simulink model "GuytonModel1972_R2018"  (R2018a)
settings: Solver=ode23tb  StartTime=0.0  StopTime=2e6  MaxStep=90  RelTol=1e-3  EnableMultiTasking=on
(part 1 of 2)
settings Model: Creator=Jirka  LastModifiedBy=User
settings SolverCC: ZeroCrossAlgorithm=Adaptive  SolverResetMethod=Robust
settings DataIOCC: LimitDataPoints=on  SaveFormat=Array
settings OptimizationCC: ExpressionDepthLimit=2147483647  InitFltsAndDblsToZero=on  LifeSpan=inf
settings DebuggingCC: SaveWithParameterizedLinksMsg=none  UnderspecifiedInitializationDetection=Classic  MergeDetectMultiDrivingBlocksExec=none  SignalResolutionControl=TryResolveAllWithWarning  MaxConsecutiveZCsMsg=warning  SolverPrmCheckMsg=warning  MultiTaskDSMMsg=warning  MultiTaskCondExecSysMsg=none  FcnCallInpInsideContextMsg=warning  StateNameClashWarn=warning  SFUnexpectedBacktrackingDiag=warning  SFNoUnconditionalDefaultTransitionDiag=warning  SFExecutionAtInitializationDiag=none
settings HardwareCC: ProdBitPerPointer=32  ProdBitPerSizeT=32  ProdBitPerPtrDiffT=32  ProdLargestAtomicFloat=None  ProdIntDivRoundTo=Undefined  ProdEndianess=Unspecified  ProdWordSize=32  ProdHWDeviceType=32-bit Generic
settings ModelReferenceCC: PropagateSignalLabelsOutOfModel=off
settings CodeAppCC: StateflowObjectComments=on
settings GRTTargetCC: TargetFcnLib=ansi_tfl_tmw.mat  TargetLangStandard=C89/C90 (ANSI)  CombineOutputUpdateFcns=off  GRTInterface=on
settings ConfigComp: CovMetricSettings=dw  CovHtmlReporting=on  CovSaveCumulativeToWorkspaceVar=on  CovSaveSingleToWorkspaceVar=on  CovExternalEMLEnable=off

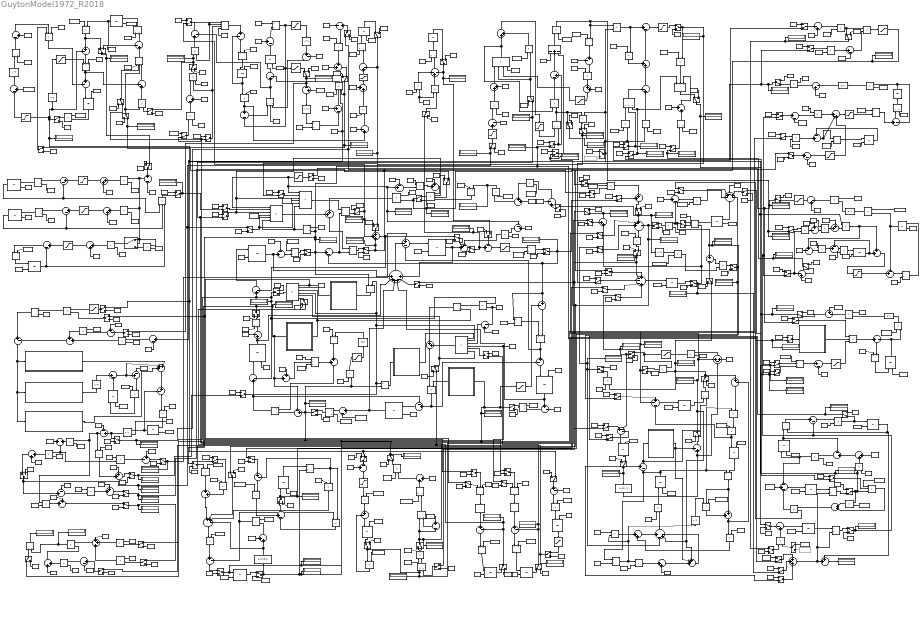
== system GuytonModel1972_R2018 ==
  note: NON-MUSCLE OXYGEN DELIVERY
  note: 269
  note: 268
  note: 261
  note: 260
  note: 270
  note: 262
  note: 263
  note: 264
  note: 271
  note: 272
  note: 265
  note: 266
  note: 267
  note: 259
  note: 258
  note: 257
  note: 256
  note: 255
  note: POV
  note: OSV
  note: POT
  note: RDO
  note: MO2
  note: DOB
  note: QO2
  note: POT
  note: P1O
  note: P4O
  note: 02M
  note: AOM
  note: 271
  note: NON-MUSCLE LOCAL BLOOD FLOW CONTROL
  note: if (POD<0) {POJ=PODx3.3}
  note: 278
  note: 277
  note: 276
  note: 275
  note: 274
  note: 273
  note: 285
  note: 282
  note: 281
  note: 280
  note: 279
  note: 290
  note: 284
  note: 283
  note: 284b
  note: 286
  note: 287
  note: 288
  note: 289
  note: AR1
  note: A1K
  note: POB
  note: POK
  note: POD
  note: POV
  note: ARM
  note: AR1
  note: AR3
  note: PON
  note: POA
  note: A2K
  note: AR2
  note: POJ
  note: POZ
  note: POC
  note: A3K
  note: AR3
  note: POR
  note: VASCULAR
      | STRESS
      | RELAXATION
  note: 65
  note: 64
  note: 63
  note: 62
  note: 61
  note: VV7
  note: VV7
  note: VV1
  note: VV2
  note: VVE
  note: VV6
  note: 195
  note: 196
  note: 197
  note: 198
  note: 199
  note: 200
  note: 201
  note: 202
  note: 203
  note: 205
  note: 206
  note: 207
  note: 208
  note: 209
  note: 210
  note: 211
  note: 212
  note: 213
  note: 214
  note: 215
  note: 216
  note: 217
  note: 218
  note: 219
  note: 220
  note: 221
  note: 222
  note: KIDNEY DYNAMICS AND EXCRETION
  note: THIRST AND DRINKING
  note: 192
  note: 193
  note: 194
  note: 190
  note: 191
  note: STH
  note: TVD
  note: POT
  note: ANTIDIURECTIC HORMONE CONTROL
  note: 181
  note: 180
  note: 179
  note: 178
  note: 177
  note: 175
  note: 176
  note: 182
  note: 183
  note: 184
  note: 185
  note: 158A
  note: 186
  note: 187
  note: 188
  note: 189
  note: AHM
  note: AH4
  note: AH2
  note: AH1
  note: AHC
  note: AH
  note: CNZ
  note: CNA
  note: PRA
  note: AHZ
  note: AH7
  note: AHY
  note: AH8
  note: AU
  note: CIRCULATORY DYNAMICS
  note: VIM
  note: AUM
  note: AUM
  note: VIM
  note: AUM
  note: BFN
  note: 1
  note: 2
  note: 3
  note: 4
  note: 36
  note: 35
  note: 31
  note: 32
  note: 33
  note: PGS
  note: RSM
  note: 38
  note: 34
  note: 37
  note: RVS
  note: 43
  note: 42
  note: 41A
  note: 41
  note: 40
  note: 39
  note: VBD
  note: VVE
  note: 5
  note: 6
  note: 7
  note: 8
  note: 9
  note: DAS
  note: QAO
  note: 30
  note: QLO
  note: LVM
  note: HPL
  note: HMD
  note: QLN
  note: 29
  note: 59
  note: 58
  note: 28
  note: 50
  note: 16
  note: PA2
  note: 60
  note: PLA
  note: 24
  note: 25
  note: 26
  note: 27
  note: VVS
  note: QLO
  note: AUH
  note: HMD
  note: QRO
  note: QRO
  note: AUH
  note: VPE
  note: PPA
  note: PL1
  note: PPA
  note: RPV
  note: RPT
  note: RPT
  note: PP1
  note: 54
  note: 53
  note: 55
  note: 56
  note: 57
  note: 52
  note: 51
  note: 23
  note: 22
  note: 21
  note: 20
  note: 19
  note: 18
  note: 48
  note: 49
  note: 46
  note: 45
  note: 47
  note: 44
  note: 10
  note: 11
  note: 12
  note: 13
  note: 14
  note: 15
  note: LVM
  note: CAPILLARY MEMBRANE DYNAMICS
  note: 66
  note: 67
  note: 68
  note: 69
  note: 70
  note: 71
  note: 74
  note: 73
  note: 82
  note: 81
  note: 80
  note: 79
  note: 78
  note: 77
  note: 75
  note: 76
  note: 72
  note: RVS
  note: BFN
  note: PVG
  note: PVS
  note: VB
  note: VP
  note: VRC
  note: PTC
  note: PPC
  note: PIF
  note: VPD
  note: VUD
  note: DFP
  note: TVD
  note: VP
  note: CPI
  note: CP1
  note: CPP
  note: CPP
  note: PRP
  note: VP
  note: CPR
  note: DLP
  note: PPD
  note: DPL
  note: DPP
  note: DPC
  note: ANGIOTENSIN CONTROL
  note: 154
  note: 157
  note: 158
  note: 159
  note: 160
  note: 161
  note: 162
  note: 163
  note: block 153
  note: block 153
  note: CNA
  note: CNE
  note: ANT
  note: ANC
  note: AN2
  note: AN3
  note: AN5
  note: ANM
  note: REK
  note: GFN
  note: TISSUE FLUIDS, PRESSURES AND GEL
  note: 105
  note: PTC
  note: 108
  note: 107
  note: 106
  note: 109
  note: 104
  note: 110
  note: 103
  note: 102
  note: 112
  note: 113
  note: 98
  note: 97
  note: 96
  note: 99
  note: 92
  note: 91
  note: 90
  note: 89
  note: 93
  note: 94
  note: 95
  note: 100
  note: 101
  note: 86
  note: 85
  note: 84
  note: 83
  note: 87
  note: 88
  note: 111
  note: DPL
  note: VTL
  note: CPI
  note: PIF
  note: PLD
  note: PTT
  note: GP1
  note: GPD
  note: GPR
  note: VG
  note: VIF
  note: PTS
  note: PIF
  note: GPD
  note: DPL
  note: VTC
  note: VTL
  note: VID
  note: VTS
  note: VTD
  note: PTT
  note: DPI
  note: VIF
  note: IFP
  note: GP2
  note: VGD
  note: VG
  note: V2D
  note: PG2
  note: PGC
  note: PTC
  note: PIF
  note: PIF
  note: PTS
  note: PRM
  note: CHY
  note: HYL
  note: VG
  note: PGR
  note: PGP
  note: PGH
  note: ALDOSTERONE CONTROL
  note: 165
  note: 166
  note: 167
  note: 164
  note: 168
  note: 169
  note: 170
  note: 171
  note: 172
  note: 173
  note: 174
  note: AM
  note: AM5
  note: AM3
  note: AM2
  note: AMC
  note: AMT
  note: AM1
  note: AMP
  note: KN1
  note: CKE
  note: CNA
  note: ANM
  note: AMR
  note: ELECTROLYTES AND CELL WATER
  note: 114
  note: 115
  note: 116
  note: 117
  note: 118
  note: 119
  note: 120
  note: 121
  note: 126
  note: 125
  note: 122
  note: 123
  note: 124
  note: 127
  note: 128
  note: 129
  note: 130
  note: 131
  note: 135
  note: 134
  note: 133
  note: 132
  note: CKI
  note: CCD
  note: CNA
  note: VIC
  note: VID
  note: VIC
  note: KI
  note: KCD
  note: KIE
  note: KIR
  note: KE1
  note: AM
  note: CKE
  note: KE
  note: KED
  note: KCD
  note: KID
  note: KOD
  note: REK
  note: NED
  note: NAE
  note: CNA
  note: VTW
  note: VIC
  note: VEC
  note: STH
  note: NID
  note: VP
  note: VPF
  note: VTS
  note: HEART HYPERTROPHY OR DETERIORATION
  note: 340
  note: 341
  note: 342
  note: 343
  note: 344
  note: 349
  note: 348
  note: 347
  note: 346
  note: 345
  note: 350
  note: 351
  note: 352
  note: PA
  note: PPA4
  note: HPL
  note: HPR
  note: PP3
  note: PPA
  note: HSL
  note: HSR
  note: POT
  note: DHM
  note: HMD
  note: RED CELLS AND VISCOSITY
  note: 329
  note: 330
  note: 331
  note: 332
  note: 333
  note: 334
  note: 335
  note: 337
  note: 338
  note: 339
  note: POT
  note: PO2
  note: RC1
  note: RCD
  note: VRC
  note: RKC
  note: RC2
  note: VRC
  note: VB
  note: HM
  note: VIE
  note: VIM
  note: PULMONARY DYNAMICS AND FLUIDS
  note: PLA
  note: 136
  note: 137
  note: 138
  note: 139
  note: 140
  note: 141
  note: 142
  note: 143
  note: 144
  note: 145
  note: 152
  note: 146
  note: 147
  note: 148
  note: 149
  note: 150
  note: 151
  note: PPA
  note: PCP
  note: PPC
  note: POS
  note: PPI
  note: PFI
  note: PLF
  note: DFP
  note: VPF
  note: PPI
  note: PLF
  note: PLF
  note: PPO
  note: POS
  note: CPN
  note: VPF
  note: PPR
  note: PPD
  note: PPN
  note: PPC
  note: CPP
  note: AUTONOMIC CONTROL
  note: 292
  note: 291
  note: 294
  note: 293
  note: 296
  note: 297
  note: 298
  note: 295
  note: 307
  note: 303
  note: 302
  note: 301
  note: 305
  note: 304
  note: 308
  note: 309
  note: 310
  note: 311
  note: 312
  note: 313
  note: 315
  note: 314
  note: 316
  note: 317
  note: 318
  note: 319
  note: 320
  note: POQ
  note: POT
  note: PA
  note: EXE
  note: EX1
  note: P2O
  note: Z12
  note: EXC
  note: AUC
  note: PA1
  note: A1B
  note: AUB
  note: AUN
  note: AU8
  note: AUK
  note: AU2
  note: AU6
  note: DAU
  note: AUJ
  note: AUO
  note: VVR
  note: AUH
  note: AUM
  note: AVE
  note: AUR
  note: AUO
  note: AU9
  note: AU
  note: HEART RATE AND STROKE VOLUME
  note: 328
  note: 327
  note: 323
  note: 322
  note: 321
  note: 324
  note: 325
  note: 326
  note: SVO
  note: QLO
  note: HR
  note: PRA
  note: AUR
  note: HMD
  note: MUSCLE BLOOD FLOW CONTROL AND PO2
  note: 227
  note: 226
  note: 225
  note: 224
  note: 223
  note: 228
  note: 229
  note: 230
  note: 231
  note: 232
  note: 233
  note: 234
  note: 235
  note: 238
  note: 236
  note: 237
  note: 239
  note: 240
  note: 241
  note: 242
  note: 243
  note: 244
  note: 245
  note: 246
  note: 247
  note: 248
  note: 249
  note: 250
  note: 251
  note: 252
  note: 253
  note: 254
  note: OSA
  note: OVA
  note: BFM
  note: RMO
  note: BFM
  note: PK1
  note: PK2
  note: OVS
  note: PVO
  note: PMO
  note: PM5
  note: RMO
  note: QOM
  note: PMO
  note: PM3
  note: PK3
  note: PM4
  note: P2O
  note: P3O
  note: EXC
  note: AOM
  note: O2A
  note: AU
  note: AMM
  note: POE
  note: POM
  note: PDO
  note: PVO
  note: POV
  note: POT
  note: ARM
  note: OVA
  note: P2O
  note: AOM
  note: AMM
  note: AMM
  note: VVE
  note: VV7
  note: VUD
  note: RBF
  note: RFN
  note: NOD
  note: AU
  note: VVR
  note: AUH
  note: AUM
  note: AVE
  note: SVO
  note: HM
  note: BFN
  note: VPF
  note: HM
  note: OVA
  note: PPC
  note: REK
  note: CNE
  note: AUM
  note: AHM
  note: AM
  note: AHM
  note: PA
  note: NOD
  note: DPC
  note: ARM
  note: VIM
  note: AUM
  note: ANM
  note: AVE
  note: RBF
  note: CN3
  note: VVR
  note: VV7
  note: AUH
  note: HMD
  note: HPR
  note: STH
  note: TVD
  note: VTL
  note: AHM
  note: CNE
  note: AM
  note: VID
  note: CKE
  note: CNA
  note: VTW
  note: PC
  note: VB
  note: VP
  note: DPC
  note: CPP
  note: VTC
  note: VTL
  note: DPL
  note: PTC
  note: CPI
  note: VTS
  note: PIF
  note: HPR
  note: HPL
  note: HMD
  note: VIM
  note: HM
  note: VRC
  note: DFP
  note: VPF
  note: PPD
  note: BFN
  note: BFM
  note: RVS
  note: PVS
  note: PRA
  note: QLO
  note: PLA
  note: PPA
  note: PA
  note: HSL
  note: PPC
  note: VTC
  note: PC
  note: GP3
  note: APD
  note: AAR-afferent arteriolar resistance [torr/l/min]
      | AHM-antidiuretic hormone multiplier, ratio of normal effect
      | AM-aldosterone multiplier, ratio of normal effect
      | AMC-aldosterone concentration
      | AMM-muscle vascular constriction caused by local tissue control, ratio to resting state
      | AMP-effect of arterial pressure on rate of aldosterone secretion
      | AMR-effect of sodium to potassium ratio on aldosterone secretion rate
      | AMT-time constant of aldosterone accumulation and destruction
      | ANC-angiotensin concentration
      | ANM-angiotensin multiplier effect on vascular resistance, ratio to normal
      | ANN-effect of sodium concentration on rate of angiotensin formation
      | ANP-effect of renal blood flow on angiotensin formation
      | ANT-time constant of angiotensin accumulation and destruction
      | ANU-nonrenal effect of angiotensin
      | AOM-autonomic effect on tissue oxygen utilization
      | APD-afferent arteriolar pressure drop [torr]
      | ARF-intensity of sympathetic effects on renal function
      | ARM-vasoconstrictor effect of all types of autoregulation
      | AR1-vasoconstrictor effect of rapid autoregulation
      | AR2-vasoconstrictor effects of intermediate autoregulation
      | AR3-vasoconstrictor effect of long-term autoregulation
      | AU-overall activity of autonomic system, ratio to normal
      | AUB-effect of baroreceptors on autoregulation
      | AUC-effect of chemoreceptors on autonomic stimulation
      | AUH-autonomic stimulation of heart, ratio to normal
  note: DLP-rate of formation of plasma protein by liver [g/min]
      | DOB-rate of oxygen delivery to non-muscle cells [ml O2/min]
      | DPA-rate of increase in pulmonary volume [l/min]
      | DPC-rate of loss of plasma proteins through systemic capillaries [g/min]
      | DPI-rate of change of protein in free interstitial fluid [g/min]
      | DPL-rate of systemic lymphatic return of protein [g/min]
      | DPO -rate of loss of plasma protein [g/min]
      | DRA-rate of increase in right atrial volume [l/min]
      | DVS-rate of increase in venous vascular volume [l/min]
      | EVR-postglomerular resistance [torr/l]
      | EXC-exercise activity, ratio to activity at rest
      | EXE-exercise effect on autonomic stimulation
      | GFN-glomerular filtration rate of undamaged kidney [l/min]
      | GFR-glomerular filtration rate [l/min]
      | GLP-glomerular pressure [torr]
      | GPD-rate of increase of protein in gel  [l/min]
      | GPR-total protein in gel  [g]
      | HM-hematocrit [%]
      | HMD-cardiac depressant effect of hypoxia
      | HPL-hypertrophy effect on left ventricle
      | HPR-hypertrophy effect on heart, ratio to normal
      | HR-heart rate [beats/min]
      | HSL-basic left ventricular strength
      | HSR-basic strength of right ventricle
      | HYL-quantity of hyaluronic acid in tissues [g]
      | IFP-interstitial fluid protein [g]
      | KCD-rate of change of potassium concentration [mmol/min]
      | KE-total extracellular fluid potassium [mmol]
      | KED-rate of change of extracellular fluid potassium concentration [mmol/min]
      | KI-total intracellular potassium concentration [mmol/l]
  note: KID-rate of potassium intake [mmol/min]
      | KOD-rate of renal loss of potassium [mmol/min]
      | LVM-effect of aortic pressure on left ventricular output
      | MMO-rate of oxygen utilization by muscle cells [ml/min]
      | M02--rate of oxygen utilization by non-muscle cells [ml/min]
      | NAE-total extracellular sodium [mmol]
      | NED-rate of change of sodium in intracellular fluids [mmol/min]
      | NID-rate of sodium intake [mmol/min]
      | NOD-rate of renal excretion of sodium [mmol/min]
      | OMM-muscle oxygen utilization at rest [ml/min]
      | OSA-aortic oxygen saturation
      | OSV-non-muscle venous oxygen saturation
      | OVA-oxygen volume in aortic blood [ml O2/l blood]
      | OVS-muscle venous oxygen saturation
      | O2M-basic oxygen utilization in non-muscle body tissues [ml/min]
      | PA-aortic pressure  [torr]
      | PAM-effect of arterial pressure in distending arteries, ratio to normal
      | PC-capillary pressure  [torr]
      | PCD-net pressure gradient across capillary membrane  [torr]
      | POP-pulmonary capillary pressure  [torr]
      | PDO-difference between muscle venous oxygen PO2 and normal venous oxygen PO2  [torr]
      | PFI-rate of transfer of fluid across pulmonary capillaries [l/min]
      | PFL-renal filtration pressure  [torr]
      | PGC-colloid osmotic pressure of tissue gel  [torr]
      | PGH-absorbency effect of gel caused by recoil of gel reticulum  [torr]
      | PGL-pressure gradient in lungs  [torr]
      | PGP-colloid osmotic pressure of tissue gel caused by entrapped protein  [torr]
      | PGR-colloid osmotic pressure of interstitial gel caused by Donnan equilibrium  [torr]
      | PIF-interstitial fluid pressure  [torr]
      | PLA-left atrial pressure  [torr]
  note: PLD-pressure gradient to cause lymphatic flow  [torr]
      | PLF-pulmonary lymphatic flow  [torr]
      | PMO-muscle cell PO2  [torr]
      | POD-non-muscle venous PO2 minus normal value  [torr]
      | POK-sensitivity of rapid system of autoregulation
      | PON-sensitivity of intermediate autoregulation
      | POS-pulmonary interstitial fluid colloid osmotic pressure  [torr]
      | POT-non-muscle cell PO2  [torr]
      | POV-non-muscle venous PO2 [torr]
      | POY-sensitivity of red cell production
      | POZ-sensitivity of long-term autoregulation
      | PO2-oxygen deficit factor causing red cell production
      | PPA-pulmonary arterial pressure  [torr]
      | PPC-plasma colloid osmotic pressure  [torr]
      | PPD-rate of change of protein in pulmonary fluids
      | PPI-pulmonary interstitial fluid pressure  [torr]
      | PPN-rate of pulmonary capillary protein loss [g/min]
      | PPO-pulmonary lymph protein flow [g/min]
      | PPR-total protein in pulmonary fluids [g]
      | PRA-right atrial pressure  [torr]
      | PRM-pressure caused by compression of interstitial fluid gel reticulum [torr]
      | PRP-total plasma protein [g]
      | PTC-interstitial fluid colloid osmotic pressure  [torr]
      | PTS-solid tissue pressure  [torr]
      | PTT-total tissue pressure  [torr]
      | PGV-pressure from veins to right atrium  [torr]
      | PVG-venous pressure gradient  [torr]
      | PVO-muscle venous PO2  [torr]
      | PVS-average venous pressure  [torr]
      | QAO-blood flow in the systemic arterial system [l/min]
  note: QLN-basic left ventricular output [l/min]
      | QLO-output of left ventricle [l/min]
      | QOM-total volume of oxygen in muscle cells [ml]
      | QO2-non-muscle total cellular oxygen [ml]
      | QPO-rate of blood flow into pulmonary veins and left atrium [l/min]
      | QRF-feedback effect of left ventricular function on right ventricular function
      | QRN-basic right ventricular output [l/min]
      | QRO-actual right ventricular output [l/min]
      | QVO-rate of blood flow from veins into right atrium [l/min]
      | RAM-basic vascular resistance of muscles [torr/l/min]
      | RAR-basic resistance of non-muscular and non-renal arteries [torr/l/min]
      | RBF-renal blood flow [l/min]
      | RC1-red cell production rate [l/min]
      | RC2-red cell destruction rate [l/min]
      | RCD-rate of change of red cell mass [l/min]
      | REK-percent of normal renal function
      | RFN-renal blood flow if kidney is not damaged [l/min]
      | RKC-rate factor for red cell destruction
      | RM0-rate of oxygen transport to muscle cells [ml/min]
      | RPA-pulmonary arterial resistance [torr/l/min]
      | RPT-pulmonary vascular resistance [torr/l/min]
      | RPV-pulmonary venous resistance [torr/l/min]
      | RR-renal resistance [torr/l/min]
      | RSM-vascular resistance in muscles [torr/l/min]
      | RSN-vascular resistance in non-muscle, non-renal tissues [torr/l/min]
      | RVG-resistance from veins to right atrium [torr/l/min]
      | RVM-depressing effect on right ventricle of pulmonary arterial pressure
      | RVS-venous resistance [torr/l/min]
      | SR-intensity factor for stress relaxation
      | SRK-time constant for stress relaxation
  note: STH-effect of tissue hypoxia on salt and water intake
      | SVO-stroke volume output [l]
      | TRR-tubular reabsorption rate [l/min]
      | TVD-rate of drinking [l/min]
      | VAS-volume in systemic arteries [l]
      | VB-blood volume [l]
      | VEC-extracellular fluid volume [l]
      | VG-volume of interstitial fluid gel [l]
      | VGD-rate of change of tissue gel volumes [l/min]
      | VIB-blood viscosity, ratio to that of water
      | VIC-cell volume [l]
      | VID-rate of fluid transfer between interstitial fluid and cells [l/min]
      | VIE-portion of blood viscosity caused by red blood cells
      | VIF-volume of free interstitial fluid [l]
      | VIM-blood viscosity (ratio to normal blood)
      | VLA-volume in left atrium [l]
      | VP-plasma volume [l]
      | VPA-volume in pulmonary arteries [l]
      | VPD-rate of change of plasma volume [l]
      | VPF-pulmonary free fluid volume [l]
      | VRA-right atrial volume [l]
      | VTC-rate of fluid transfer across systemic capillary membranes [l/min]
      | VTD-rate of volume change in total interstitial fluid [l/min]
      | VTL-rate of systemic lymph flow [l/min]
      | VTW-total body water [l]
      | VUD-rate of urinary output [l/min]
      | VV7-increased vascular volume caused by stress relaxation [l]
      | VVR-diminished vascular volume caused by sympathetic stimulation [l]
      | VVS-venous vascular volume [l]
      | Z8-time constant of autonomic response
  note: AUK-time constant of baroreceptor adaptation
      | AUL-sensitivity of sympathetic control of vascular capacitance
      | AUM-sympathetic vasoconstrictor effect on arteries
      | AUN-effect of CNS ischemic reflex on auto-regulation
      | AUV-sensitivity control of autonomies on heart function
      | AUY-sensitivity of sympathetic control of veins
      | AUZ-overall sensitivity of autonomic control
      | AVE-sympathetic vasoconstrictor effect on veins
      | AlK-time constant of rapid autoregulation
      | A2K-time constant of intermediate autoregulation
      | A3K-time constant of long-term autoregulation
      | A4K-time constant for muscle local vascular response to metabolic activity
      | BFM-muscle blood flow [l/min]
      | BFN-blood flow in non-muscle, non-renal tissues [l/min]
      | CA-capacitance of systemic arteries [l/torr]
      | CCD-concentration gradient across cell membrane [mmol/l]
      | CHY-concentration of hyaluronic acid in tissue fluids [g/l]
      | CKE-extracellular potassium concentration [mmol/l]
      | CKI-intracellular potassium concentration [mmol/l]
      | CNA-extracellular sodium concentration [mmol/l]
      | CNE-sodium concentration abnormality causing third factor effect [mmo/l]
      | CPG-concentration of protein in tissue gel [g/l]
      | CPI-concentration of protein in free interstitial fluid [g/l]
      | CPN-concentration of protein in pulmonary fluids [g/l]
      | CPP-plasma protein concentration [g/l]
      | CV-venous capacitance [l/torr]
      | DAS-rate of volume increase of systemic arteries [l/min]
      | DFP-rate of increase in pulmonary free fluid [l/min]
      | DHM-rate of cardiac deterioration caused by hypoxia
      | DLA-rate of volume increase in pulmonary veins and left atrium [l/min]
  note: LIST OF VARIABLES
  note: 336
  note: HM2
  note: 336b
  note: HMK
  note: HR
  note: PA
  note: OMM
  note: PA0
  note: 299
  note: 300
  note: 306
  note: HR
  note: HRN
  note: HRPRA
  note: HRAU
  note: HRHMD
  note: HKM
  note: VIB
  note: PVG
  note: RDNORM
  note: 17
  note: DPA
  note: RSNA
  note: RSNV
  note: QRRF
  note: FQLN
  note: FQRN
  note: RVV7
  note: CPPK
  note: LPD
  note: PGH
  note: CPG
  note: PHYX
  note: PGX
  note: PC
  note: VIM
  note: AGK
  note: ANW
  note: ANR
  note: ANV
  note: ANP
  note: AN1
  note: 155-156
  note: AU
  note: AUP
  note: AUR
  note: AUR
  note: 315a
  note: 312B
  note: 312A
  " lower limit 0" : Saturate  UpperLimit=inf  LowerLimit=0.0001  LinearizeAsGain=off
  " lower limit 0.35" : Saturate  UpperLimit=inf  LowerLimit=0.35  LinearizeAsGain=off
   VAS{,1..5} (6 alike) : Integrator  InitialConditionSource=external
  " VLA" : Integrator  InitialConditionSource=external
  " VPA" : Integrator  InitialConditionSource=external
  " VRA" : Integrator  InitialConditionSource=external
  " VVS" : Integrator  InitialConditionSource=external
  "1 " : Constant
  AMP = f(PA) : Subsystem
      mask Display:
      | plot([ 0    10    20    30    40    50    60    70    80    90   100   110   120   130   140   150   160   170   180   190   200], [4.0000    3.6505    3.3040    2.9635    2.6320    2.3125    2.0080    1.7215    1.4560    1.2145    1.0000    0.8145    0.6560    0.5215    0.4080    0.3125    0.2320    0.1635    0.1040    0.0505    0.0000])
      | 
      | text(-20,2,'')
      | text(230,2,'')
      | text(100,4.2,'')
      | text(100,-0.4,'')
      | 
      | text(-16,0,'0')
      | text(0,-0.2,'0')
      | text(-16,4,'4')
      | text(190,-0.2,'200')
  ANY : Constant  Value=0.2
  ANZ : Constant  Value=0.4
  ARF : Constant  Value=1.5
  AUB calculation : Subsystem
      mask Display: disp('AUB CALCULATION \n\nwhen PA1<40: AUB=1.85718             \nwhen  40>PA1<170: AUB=0.014286*(170-PA1)\nwhen PA1>=170: AUB=0               \n')
  AUB^3 : Fcn  Expr=u^3
  AUC calculation : Subsystem
      mask Display: disp('AUC CALCULATION \n\nwhen PA1<40: AUC=1.2             \nwhen  40>PA1<80: AUC=0.03*(80-PA1)\nwhen PA1>=80: AUC=0               \n')
  AUJ^AUZ : Math  Operator=pow  SaturateOnIntegerOverflow=on
  AUL : Constant  Value=0.21
  AUN calculation : Subsystem
      mask Display: disp('AUN CALCULATION \n\nwhen PA1<50: AUN=6            \nwhen  20>PA1<50: AUN=0.2*(50-PA1)\nwhen PA1>=50: AUN=0               \n')
  AUQ : Constant
  AUS : Constant
  AUV : Constant  Value=0.3
  AUY : Constant  Value=0.5
  AUZ : Constant
  CFC : Constant  Value=0.007
  CHY^2 : Fcn  Expr=u^2
  CN2 : Constant  Value=0.0212
  CN7 : Constant  Value=0.2
  CNR : Constant  Value=139
  CNX : Constant  Value=2.5
  CNY : Constant  Value=6
  CPF : Constant  Value=0.0003
  CPK : Constant  Value=1.6283e-007
  CV : Constant  Value=0.0825
  Constant{1,14,16,18..20,22..24,27,29,35,45..47,54,58,61,67,76,78,94,137,149..150,153..155,158,160,166,169,171,175..176,183,189..191,195..196,198..201,205,209,213,216,234..235,241,244..249,254..257,260,274,280,282..283,285,295..297,299,304..306,308..309,322,327..328,330..331,334..335} (84 alike) : Constant
  Constant{7..8,10,172,178,211,229,237,258,267,287,290,315,324} (14 alike) : Constant  Value=5
  Constant100 : Constant  Value=0.013332
  Constant101 : Constant  Value=0.25
  Constant102 : Constant  Value=7.8
  Constant103 : Constant  Value=0.004
  Constant{63..64,85,104,116,215,277} (7 alike) : Constant  Value=0.1
  Constant{82..83,86,105,146} (5 alike) : Constant  Value=0.4
  Constant106 : Constant  Value=57
  Constant107 : Constant  Value=-5.9
  Constant108 : Constant  Value=24.2
  Constant109 : Constant  Value=0.25
  Constant11 : Constant  Value=-1
  Constant110 : Constant  Value=9
  Constant111 : Constant  Value=60
  Constant112 : Constant  Value=-0.0391
  Constant113 : Constant  Value=19.8
  Constant114 : Constant  Value=20.039
  Constant115 : Constant  Value=0.00352
  Constant117 : Constant  Value=0.00042
  Constant118 : Constant  Value=0.00014
  Constant119 : Constant  Value=0.0028
  Constant12 : Constant  Value=8.0001
  Constant120 : Constant  Value=0.013
  Constant121 : Constant  Value=140
  Constant122 : Constant  Value=0.01
  Constant123 : Constant  Value=2850
  Constant{62,124,132,193,210,223,238,323} (8 alike) : Constant  Value=100
  Constant125 : Constant  Value=57600
  Constant{95,126,224,230,326} (5 alike) : Constant  Value=15
  Constant127 : Constant  Value=57600
  Constant128 : Constant  Value=6
  Constant129 : Constant  Value=0.0025
  Constant13 : Constant  Value=512
  Constant131 : Constant  Value=0.0000058
  Constant134 : Constant  Value=0.5333
  Constant135 : Constant  Value=1.5
  Constant136 : Constant  Value=0.333
  Constant138 : Constant  Value=0.55
  Constant{139,187,217,301} (4 alike) : Constant  Value=0.0125
  Constant140 : Constant  Value=0.4667
  Constant142 : Constant  Value=11
  Constant143 : Constant  Value=0.0003
  Constant144 : Constant  Value=0.000225
  Constant145 : Constant  Value=0.375
  Constant{147,157,204,214,226..228,239..240} (9 alike) : Constant  Value=8
  Constant15 : Constant  Value=60
  Constant151 : Constant  Value=0.15
  Constant152 : Constant  Value=0.85
  Constant{56,156,218,310} (4 alike) : Constant  Value=3
  Constant159 : Constant  Value=1.24
  Constant161 : Constant  Value=0.0005
  Constant164 : Constant  Value=2
  Constant{25,165,174,184,188,206,243,300} (8 alike) : Constant  Value=40
  Constant167 : Constant  Value=0.5
  Constant168 : Constant  Value=32
  Constant17 : Constant  Value=0.15
  Constant170 : Constant  Value=0.025
  Constant173 : Constant  Value=0.08
  Constant177 : Constant  Value=0.5
  Constant179 : Constant  Value=57.14
  Constant180 : Constant  Value=122
  Constant181 : Constant  Value=2500
  Constant182 : Constant  Value=800
  Constant185 : Constant  Value=2.8
  Constant186 : Constant  Value=200
  Constant{30..31,192,319} (4 alike) : Constant  Value=0.3
  Constant194 : Constant  Value=28
  Constant{197,284,332..333} (4 alike) : Constant  Value=10
  Constant2 : Constant  Value=168
  Constant{202,221,231,236,253,268,271,275,286,302..303,320,325} (13 alike) : Constant  Value=0
  Constant{203,207,212,288} (4 alike) : Constant  Value=142
  Constant208 : Constant  Value=0.125
  Constant21 : Constant  Value=11520
  Constant219 : Constant  Value=12
  Constant{220,270,291,313} (4 alike) : Constant  Value=0.002
  Constant{222,273,292,312} (4 alike) : Constant  Value=0.04
  Constant225 : Constant  Value=200
  Constant232 : Constant  Value=28
  Constant233 : Constant  Value=70
  Constant250 : Constant  Value=1.2
  Constant{68..69,251,314} (4 alike) : Constant  Value=17
  Constant252 : Constant  Value=2.95
  Constant26 : Constant  Value=0.06
  Constant{38,261,269,276} (4 alike) : Constant  Value=0.001
  Constant262 : Constant  Value=2.9
  Constant263 : Constant  Value=2.8
  Constant264 : Constant  Value=3.7
  Constant265 : Constant  Value=2
  Constant266 : Constant  Value=-6.3
  Constant{28,74,272,294} (4 alike) : Constant  Value=20
  Constant278 : Constant  Value=1.2
  Constant279 : Constant  Value=1.2
  Constant281 : Constant  Value=17.75
  Constant289 : Constant  Value=12
  Constant293 : Constant  Value=-6.3
  Constant298 : Constant  Value=2
  Constant3 : Constant  Value=2688
  Constant307 : Constant  Value=2.95
  Constant311 : Constant  Value=70
  Constant316 : Constant  Value=28
  Constant317 : Constant  Value=3.7
  Constant318 : Constant  Value=2.9
  Constant32 : Constant  Value=0.301
  Constant321 : Constant  Value=2.8
  Constant329 : Constant  Value=0.2
  Constant33 : Constant  Value=0.5
  Constant36 : Constant  Value=0.8
  Constant37 : Constant  Value=1000
  Constant39 : Constant  Value=0.025
  Constant4 : Constant  Value=8.0001
  Constant40 : Constant  Value=31.67
  Constant41 : Constant  Value=51.66
  Constant42 : Constant  Value=18
  Constant43 : Constant  Value=0.00781
  Constant44 : Constant  Value=0.125
  Constant48 : Constant  Value=0.01
  Constant49 : Constant  Value=0.009
  Constant5 : Constant  Value=57.14
  Constant52 : Constant  Value=6
  Constant53 : Constant  Value=7
  Constant55 : Constant  Value=-0.1808
  Constant59 : Constant  Value=0.2
  Constant6 : Constant  Value=0.00333
  Constant60 : Constant  Value=1440
  Constant65 : Constant  Value=0.005
  Constant66 : Constant  Value=0.38
  Constant70 : Constant  Value=3.25
  Constant71 : Constant  Value=0.30625
  Constant72 : Constant  Value=0.0048
  Constant73 : Constant  Value=0.85
  Constant75 : Constant  Value=0.0357
  Constant77 : Constant  Value=0.026
  Constant79 : Constant  Value=2.738
  Constant80 : Constant  Value=0.495
  Constant81 : Constant  Value=0.00355
  Constant84 : Constant  Value=1.79
  Constant9 : Constant  Value=512
  Constant90 : Constant  Value=85
  Constant92 : Constant  Value=1.79
  Constant93 : Constant  Value=152
  Constant96 : Constant  Value=-0.0967
  Constant97 : Constant  Value=3.3
  Constant98 : Constant  Value=4.0
  Constant99 : Constant  Value=0.0005
  DP0 : Constant  Value=0.007
  Display{1..76} (76 alike) : Display
  From Workspace : FromWorkspace  Commented=on  VariableName=NID_input  OutDataTypeStr=double  SampleTime=0  Interpolate=off  OutputAfterFinalValue=Holding final value
  From Workspace1 : FromWorkspace  Commented=on  VariableName=REK_input  OutDataTypeStr=double  SampleTime=0  Interpolate=off  OutputAfterFinalValue=Holding final value
  GF4 : Constant  Value=5
  HSR : Constant
  IFP0 : Constant  Value=12
  Integrator : Integrator
  Integrator QO{1..2,5..7} (5 alike) : Integrator  InitialConditionSource=external  InitialCondition=2403.143066
  Integrator1 : Integrator  InitialConditionSource=external
  Integrator2 : Integrator  InitialCondition=1
  Integrator3 : Integrator  InitialConditionSource=external
  Integrator4 : Integrator  InitialConditionSource=external
  Integrator5 : Integrator  InitialConditionSource=external  InitialCondition=2399.9633789
  Integrator7 : Integrator  InitialConditionSource=external  InitialCondition=2399.9633789
  Integrator8 : Integrator  InitialConditionSource=external  LimitOutput=on  LowerSaturationLimit=0
  KE {,1..11,13..14} (14 alike) : Integrator  InitialConditionSource=external  InitialCondition=74.7024
  LPK : Constant  Value=0.00047
  LVM = f(PA2) : Subsystem
      mask Display:
      | plot([0 2.1 4.2 6.3 8.4 10.5 12.6 14.7 16.8 18.9 21 23.1 25.2 27.3 29.4 31.5 33.6 35.7 37.8 39.9 42 44.1 46.2 48.3 50.4 52.5 54.6 56.7 58.8 60.9 63 65.1 67.2 69.3 71.4 73.5 75.6 77.7 79.8 81.9 84 86.1 88.2 90.3 92.4 94.5 96.6 98.7 100.8 102.9 105 107.1 109.2 111.3 113.4 115.5 117.6 119.7 121.8 123.9 126 128.1 130.2 132.3 134.4 136.5 138.6 140.7 142.8 144.9 147 149.1 151.2 153.3 155.4 157.5 159.6 161.7 163.8 165.9 168 170.1 172.2 174.3 176.4 178.5 180.6 182.7 184.8 186.9 189 191.1 193.2 195.3 197.4 199.5 201.6 203.7 205.8 207.9 210 212.1 214.2 216.3 218.4 220.5 222.6 224.7 226.8 228.9 231 233.1 235.2 237.3 239.4], [1.04 1.03998 1.03993 1.03985 1.03973 1.03958 1.03941 1.0392 1.03896 1.03869 1.03839 1.03807 1.03772 1.03734 1.03693 1.03651 1.03605 1.03558 1.03508 1.03455 1.03401 1.03345 1.03286 1.03225 1.03163 1.03099 1.03033 1.02965 1.02895 1.02824 1.02752 1.02678 1.02603 1.02526 1.02443 1.0234 1.02218 1.02078 1.01923 1.01753 1.01572 1.01381 1.01181 1.00976 1.00766 1.00554 1.00341 1.00129 0.999208 0.997118 0.994998 0.992831 0.9906 0.988287 0.985875 0.983347 0.980687 0.977876 0.974898 0.971736 0.968374 0.964817 0.961055 0.95708 0.952882 0.948451 0.943777 0.93885 0.93366 0.928197 0.922452 0.916415 0.910075 0.903423 0.89645 0.889144 0.881496 0.873291 0.86413 0.854038 0.84305 0.831201 0.818528 0.805065 0.790848 0.775913 0.760295 0.744029 0.727152 0.709697 0.691702 0.673201 0.65423 0.634825 0.61502 0.594852 0.574045 0.551912 0.528467 0.503753 0.477816 0.4507 0.422449 0.393107 0.362719 0.33133 0.298983 0.265724 0.231596 0.196644 0.160913 0.124446 0.087288 0.0494838 0.0110776])
      | 
      | text(-30,0.5,'')
      | text(260,0.5,'')
      | text(25,1.15,'')
      | text(25,-0.1,'')
      | text(-25,0.05,'0')
      | text(10,-0.04,'0')
      | text(-25,1.1,'1.4')
      | text(218,-0.04,'260')
  Manual Switch{,3,7..9,12,15,18,23,31..33,40..42,46..47,49..59,63..64,68..69,74..76,80,82..88,90..93,100,103..105,107..110,113..120,122..123,125,127,129..133,135,138..140,142..143} (78 alike) : ManualSwitch
  Manual Switch{1..2,4..6,10..11,13..14,16..17,19..22,24..30,34..39,43..45,48,60..62,65..67,70..73,77..79,81,89,94..99,101..102,106,111..112,121,124,126,128,134,136..137} (65 alike) : ManualSwitch  CurrentSetting=0
  Math Function : Math  SaturateOnIntegerOverflow=on
  Math Function1 : Math  Operator=sqrt  SaturateOnIntegerOverflow=on
  Math Function2 : Math  SaturateOnIntegerOverflow=on
  Math Function3 : Math  SaturateOnIntegerOverflow=on
  P3O^3 : Fcn  Expr=u^3
  P40^3 : Fcn  Expr=u^3
  PA4^0.625 : Fcn  Expr=u^0.625
  PC^3 : Fcn  Expr=u^3
  PM1^2 : Fcn  Expr=u^2
  PO1 : Constant  Value=8.25
  POK8 : Constant  Value=0.33
  POT^3 : Fcn  Expr=u^3
  POY : Constant  Value=464e-7
  PP3^0.1 : Fcn  Expr=u^0.625
  PPI = 2 - (0.15/VPF) : Fcn  Expr=2-(0.15/u)
  PTS = f(VIF) : Subsystem
      mask Display:
      | plot([0    0.5000    1.0000    1.5000    2.0000    2.5000    3.0000    3.5000    4.0000    4.5000    5.0000    5.5000    6.0000    6.5000    7.0000    7.5000    8.0000    8.5000    9.0000    9.5000   10.0000], [19.9974    8.2145    4.9644    3.4422    2.5594    1.9830    1.5771    1.2757    1.0432    0.8583    0.7078    0.5828    0.4775    0.3874    0.3096    0.2416    0.1818    0.1287    0.0812    0.0385   0.0000 ])
      | text(0,22,'')
      | text(0,-2,'')
      | text(-0.5,10,'')
      | text(10.5,10,'')
      | text(-0.2,1,'0')
      | text(0.5,-1,'0')
      | text(-0.2,21,'20')
      | text(9.5,-1,'10')
  PTT = (VTS/12)^2 : Fcn  Expr=(u/12)^2
  Product1 : Product  Inputs=/**  SaturateOnIntegerOverflow=on  RndMeth=Zero  InputSameDT=on  OutDataTypeStr=Inherit: Same as first input
  Product10 : Product  Inputs=4  SaturateOnIntegerOverflow=on  RndMeth=Zero  InputSameDT=on  OutDataTypeStr=Inherit: Same as first input
  Product{5,9,18,84,100,110,118} (7 alike) : Product  Inputs=3  SaturateOnIntegerOverflow=on  RndMeth=Zero  InputSameDT=on  OutDataTypeStr=Inherit: Same as first input
  Product{2..3,7,11,13..15,17,19,21,23,25..26,28..33,38..41,44..47,49,52..54,60,62..63,65,74,81,83,85..88,90..92,95..96,98..99,101..102,104..105,107..108,111,113,115..117,119,121..122,127,129..130,132..133,136..141,143..150,152..157,159,165..169} (94 alike) : Product  SaturateOnIntegerOverflow=on  RndMeth=Zero  InputSameDT=on  OutDataTypeStr=Inherit: Same as first input
  Product{4,12,27,42..43,50,58,64,68..70,72,76,78,80,97,103,109,135} (19 alike) : Product  Inputs=/*  SaturateOnIntegerOverflow=on  RndMeth=Zero  InputSameDT=on  OutDataTypeStr=Inherit: Same as first input
  Product{8,16,20,22,24,35,48,56..57,59,66..67,71,75,89,93,106,114,120,123..124,126,131,134,142,151,158,161,163..164} (30 alike) : Product  Inputs=*/  SaturateOnIntegerOverflow=on  RndMeth=Zero  InputSameDT=on  OutDataTypeStr=Inherit: Same as first input
  Product{36,112,125,128} (4 alike) : Product  Inputs=/*/  SaturateOnIntegerOverflow=on  RndMeth=Zero  InputSameDT=on  OutDataTypeStr=Inherit: Same as first input
  Product160 : Product  Inputs=**/  SaturateOnIntegerOverflow=on  RndMeth=Zero  InputSameDT=on  OutDataTypeStr=Inherit: Same as first input
  Product162 : Product  Inputs=*///  SaturateOnIntegerOverflow=on  RndMeth=Zero  InputSameDT=on  OutDataTypeStr=Inherit: Same as first input
  Product34 : Product  Inputs=*//  SaturateOnIntegerOverflow=on  RndMeth=Zero  InputSameDT=on  OutDataTypeStr=Inherit: Same as first input
  Product37 : Product  Inputs=4  SaturateOnIntegerOverflow=on  RndMeth=Zero  InputSameDT=on  OutDataTypeStr=Inherit: Same as first input
  Product51 : Product  Inputs=**  SaturateOnIntegerOverflow=on  RndMeth=Zero  InputSameDT=on  OutDataTypeStr=Inherit: Same as first input
  Product{55,61,77,79} (4 alike) : Product  Inputs=6  SaturateOnIntegerOverflow=on  RndMeth=Zero  InputSameDT=on  OutDataTypeStr=Inherit: Same as first input
  Product6 : Product  Inputs=///*  SaturateOnIntegerOverflow=on  RndMeth=Zero  InputSameDT=on  OutDataTypeStr=Inherit: Same as first input
  Product73 : Product  Inputs=*//  SaturateOnIntegerOverflow=on  RndMeth=Zero  InputSameDT=on  OutDataTypeStr=Inherit: Same as first input
  Product82 : Product  Inputs=4  SaturateOnIntegerOverflow=on  RndMeth=Zero  InputSameDT=on  OutDataTypeStr=Inherit: Same as first input
  Product94 : Product  Inputs=**  SaturateOnIntegerOverflow=on  RndMeth=Zero  InputSameDT=on  OutDataTypeStr=Inherit: Same as first input
  QLN = f(PLA) : Subsystem
      mask Display:
      | plot([     -5 -4 -3 -2 -1 0 1 2 3 4 5 6 7 8 9 10 11 12 13 14 15 16 17 18 19 20], [ 0 0.01 0.65885 2.08416 3.6 5.05 6.60577 8.16154 9.4 10.2738 10.9872 11.6 12.2245 12.8412 13.3123 13.5 13.5 13.5 13.5 13.5 13.5 13.5 13.5 13.5 13.5 13.5] )
      | 
      | 
      | text(-8,10,'')
      | text(10,-1.5,'')
      | text(22,10,'')
      | text(16,16,'')
      | text(-7,1,'0')
      | text(-5,-0.8,'-4')
      | text(-7,15,'15')
      | text(18,0,'20')
  QRF : Constant  Value=0.6
  QRN = f(PRA) : Subsystem
      mask Display:
      | plot([     -6 -5 -4 -3 -2 -1 0 1 2 3 4 5 6 7 8 9 10 11 12 13 14 15 16 17 18 19 20], [0 0.103491 0.373648 0.75 1.42618 2.6 5 7.61127 9.8 11.1961 12.1 12.6396 13.0852 13.3882 13.5 13.5 13.5 13.5 13.5 13.5 13.5 13.5 13.5 13.5 13.5 13.5 13.5])
      | 
      | 
      | 
      | text(-8,10,'')
      | text(10,-1.5,'')
      | text(22,10,'')
      | text(16,16,'')
      | text(-7,1,'0')
      | text(-5,-0.8,'-4')
      | text(-7,15,'15')
      | text(18,0,'20')
  RAM : Constant  Value=96.3
  RAR : Constant  Value=30.52
  RVM = f(PP2) : Subsystem
      mask Display:
      | plot([0 2.5 5 7.5 10 12.5 15 17.5 20 22.5 25 27.5 30 32.5 35 37.5 40 42.5 45], [1.06 1.05508 1.04813 1.03961 1.03 1.01865 1.00472 0.988437 0.97 0.947748 0.915021 0.864829 0.8 0.715601 0.608483 0.485782 0.347126 0.183428 5.55112e-017])
      | 
      | text(-8,0.5,'')
      | text(50,0.5,'')
      | text(25,1.15,'')
      | text(25,-0.1,'')
      | text(-7,0.05,'0')
      | text(-2,-0.04,'0')
      | text(-7,1.1,'1.4')
      | text(44,-0.04,'50')
  SRK : Constant  Value=33
  Sum{1..2,4,6,9,22,27,37,40,42,44,47..49,53,59,71,76,92,98,111,119,125,133..134,138,141} (27 alike) : Sum  Inputs=-+|  SaturateOnIntegerOverflow=on  InputSameDT=on  OutDataTypeStr=Inherit: Same as first input
  Sum{8,10,23,31,54..56,58,64..65,75,88,105,108..109,112,136,139..140,143} (20 alike) : Sum  Inputs=++|  SaturateOnIntegerOverflow=on  InputSameDT=on  OutDataTypeStr=Inherit: Same as first input
  Sum{52,78,86,100,106,114,118,120,128,131,135,137} (12 alike) : Sum  Inputs=+-|  SaturateOnIntegerOverflow=on  InputSameDT=on  OutDataTypeStr=Inherit: Same as first input
  Sum101 : Sum  Inputs=+-  SaturateOnIntegerOverflow=on  InputSameDT=on  OutDataTypeStr=Inherit: Same as first input
  Sum102 : Sum  Inputs=||+-+-  SaturateOnIntegerOverflow=on  InputSameDT=on  OutDataTypeStr=Inherit: Same as first input
  Sum{15..16,18,21,24,28,46,82..83,93,99,103,110,121} (14 alike) : Sum  Inputs=|++  SaturateOnIntegerOverflow=on  InputSameDT=on  OutDataTypeStr=Inherit: Same as first input
  Sum{12,14,17,19,29..30,32,36,39,41,50..51,61,69,77,84,94..97,104,107,113,115,117,123..124,127,129} (29 alike) : Sum  Inputs=|+-  SaturateOnIntegerOverflow=on  InputSameDT=on  OutDataTypeStr=Inherit: Same as first input
  Sum11 : Sum  Inputs=-|+  SaturateOnIntegerOverflow=on  InputSameDT=on  OutDataTypeStr=Inherit: Same as first input
  Sum116 : Sum  Inputs=+++|  SaturateOnIntegerOverflow=on  InputSameDT=on  OutDataTypeStr=Inherit: Same as first input
  Sum122 : Sum  Inputs=+++  SaturateOnIntegerOverflow=on  InputSameDT=on  OutDataTypeStr=Inherit: Same as first input
  Sum{13,34,67,85,126} (5 alike) : Sum  Inputs=+|-  SaturateOnIntegerOverflow=on  InputSameDT=on  OutDataTypeStr=Inherit: Same as first input
  Sum{3,5,7,25,33,38,45,70,72,89,130} (11 alike) : Sum  Inputs=|-+  SaturateOnIntegerOverflow=on  InputSameDT=on  OutDataTypeStr=Inherit: Same as first input
  Sum142 : Sum  Inputs=+||+  SaturateOnIntegerOverflow=on  InputSameDT=on  OutDataTypeStr=Inherit: Same as first input
  Sum20 : Sum  Inputs=-+-  SaturateOnIntegerOverflow=on  InputSameDT=on  OutDataTypeStr=Inherit: Same as first input
  Sum26 : Sum  Inputs=-+-  SaturateOnIntegerOverflow=on  InputSameDT=on  OutDataTypeStr=Inherit: Same as first input
  Sum35 : Sum  Inputs=|||+|-+  SaturateOnIntegerOverflow=on  InputSameDT=on  OutDataTypeStr=Inherit: Same as first input
  Sum43 : Sum  Inputs=--+||  SaturateOnIntegerOverflow=on  InputSameDT=on  OutDataTypeStr=Inherit: Same as first input
  Sum57 : Sum  Inputs=+++  SaturateOnIntegerOverflow=on  InputSameDT=on  OutDataTypeStr=Inherit: Same as first input
  Sum60 : Sum  Inputs=+--  SaturateOnIntegerOverflow=on  InputSameDT=on  OutDataTypeStr=Inherit: Same as first input
  Sum62 : Sum  Inputs=++++-+  SaturateOnIntegerOverflow=on  InputSameDT=on  OutDataTypeStr=Inherit: Same as first input
  Sum63 : Sum  Inputs=+-+|-  SaturateOnIntegerOverflow=on  InputSameDT=on  OutDataTypeStr=Inherit: Same as first input
  Sum66 : Sum  Inputs=+---+  SaturateOnIntegerOverflow=on  InputSameDT=on  OutDataTypeStr=Inherit: Same as first input
  Sum68 : Sum  Inputs=-+-+-  SaturateOnIntegerOverflow=on  InputSameDT=on  OutDataTypeStr=Inherit: Same as first input
  Sum73 : Sum  Inputs=+-+  SaturateOnIntegerOverflow=on  InputSameDT=on  OutDataTypeStr=Inherit: Same as first input
  Sum74 : Sum  Inputs=+++||  SaturateOnIntegerOverflow=on  InputSameDT=on  OutDataTypeStr=Inherit: Same as first input
  Sum79 : Sum  Inputs=|+--  SaturateOnIntegerOverflow=on  InputSameDT=on  OutDataTypeStr=Inherit: Same as first input
  Sum80 : Sum  Inputs=+|-+-  SaturateOnIntegerOverflow=on  InputSameDT=on  OutDataTypeStr=Inherit: Same as first input
  Sum81 : Sum  Inputs=+--  SaturateOnIntegerOverflow=on  InputSameDT=on  OutDataTypeStr=Inherit: Same as first input
  Sum87 : Sum  Inputs=+++  SaturateOnIntegerOverflow=on  InputSameDT=on  OutDataTypeStr=Inherit: Same as first input
  Sum90 : Sum  Inputs=|++|  SaturateOnIntegerOverflow=on  InputSameDT=on  OutDataTypeStr=Inherit: Same as first input
  Sum91 : Sum  Inputs=-+-  SaturateOnIntegerOverflow=on  InputSameDT=on  OutDataTypeStr=Inherit: Same as first input
  Switch1 : Switch  Criteria=u2 > Threshold  SaturateOnIntegerOverflow=on  InputSameDT=on
  VV9 : Constant  Value=3.159
  Xo : Constant  Value=2400  VectorParams1D=off
  Xo1 : Constant  VectorParams1D=off
  Xo2 : Constant  VectorParams1D=off
  Xo3 : Constant  Value=0.7  VectorParams1D=off
  Xo5 : Constant  VectorParams1D=off
  Xo6 : Constant  Value=0  VectorParams1D=off
  Z1 : Constant  Value=0.7
  Z10 : Constant  Value=11.4
  "Z10 " : Constant  Value=8.25
  Z{11,16..18,22} (5 alike) : Constant
  "Z11 " : Constant  Value=4
  Z12 : Constant  Value=3550
  Z13 : Constant  Value=2130
  Z14 : Constant  Value=25
  Z15 : Constant  Value=75
  Z2 : Constant  Value=2400
  Z20 : Constant  Value=2
  Z21 : Constant  Value=0
  Z3 : Constant  Value=90
  Z5 : Constant  Value=210
  Z6 : Constant  Value=3
  Z7 : Constant  Value=171
  Z8 : Constant  Value=6
  Z9 : Constant  Value=12
  lower limit .001 : Saturate  UpperLimit=inf  LowerLimit=0.001  LinearizeAsGain=off
  lower limit .005 : Saturate  UpperLimit=inf  LowerLimit=0.005  LinearizeAsGain=off
  lower limit 0 : Saturate  UpperLimit=inf  LowerLimit=0  LinearizeAsGain=off
  "lower limit 0 " : Saturate  UpperLimit=inf  LowerLimit=0  LinearizeAsGain=off
  lower limit 0.0001 : Saturate  UpperLimit=inf  LowerLimit=0.0001  LinearizeAsGain=off
  lower limit 0.0003 : Saturate  UpperLimit=inf  LowerLimit=0.0003  LinearizeAsGain=off
  lower limit 0.2 : Saturate  UpperLimit=inf  LowerLimit=0.2  LinearizeAsGain=off
  lower limit 0.2375 : Saturate  UpperLimit=inf  LowerLimit=0.2375  LinearizeAsGain=off
  lower limit 0.3 : Saturate  UpperLimit=inf  LowerLimit=0.3  LinearizeAsGain=off
  lower limit 0.5 : Saturate  UpperLimit=inf  LowerLimit=0.5  LinearizeAsGain=off
  lower limit 0.7 : Saturate  UpperLimit=inf  LowerLimit=0.7  LinearizeAsGain=off
  lower limit 0.95 : Saturate  UpperLimit=inf  LowerLimit=0.95  LinearizeAsGain=off
  lower limit 3 : Saturate  UpperLimit=inf  LowerLimit=0  LinearizeAsGain=off
  lower limit 50 : Saturate  UpperLimit=inf  LowerLimit=50  LinearizeAsGain=off
  lower limit 6 : Saturate  UpperLimit=inf  LowerLimit=0  LinearizeAsGain=off
  lower limit =  0 : Saturate  UpperLimit=inf  LowerLimit=0  LinearizeAsGain=off
  lower limit = 0 : Saturate  UpperLimit=inf  LowerLimit=0  LinearizeAsGain=off
  lower limit = 0.01 upper limit =100 : Saturate  UpperLimit=100  LowerLimit=0.01  LinearizeAsGain=off
  lower_limit_0 : Saturate  UpperLimit=inf  LowerLimit=0  LinearizeAsGain=off
  upper limit 1 : Saturate  UpperLimit=1  LowerLimit=0  LinearizeAsGain=off
  upper limit 15.0 lower limit 0.4 : Saturate  UpperLimit=15  LowerLimit=0.4  LinearizeAsGain=off
  upper limit 8 : Saturate  UpperLimit=8  LowerLimit=0  LinearizeAsGain=off
  upper limit 8 lower limit 4 : Saturate  UpperLimit=8  LowerLimit=4  LinearizeAsGain=off  ZeroCross=off
  "upper limit 8  " : Saturate  UpperLimit=8  LowerLimit=-inf  LinearizeAsGain=off  ZeroCross=off
  wires:
  Product8/1 -> Sum5/1
  Constant9/1 -> Product8/2
  Constant1/1 -> Sum5/2
  Sum5/1 -> Product5/2
  Constant2/1 -> Product5/3
  Product5/1 -> Sum1/1
  Product1/1 -> Sum1/2, Sum6/1
  P40^3/1 -> Product8/1
  Constant4/1 -> Sum3/2
  Constant5/1 -> Product2/1
  Constant6/1 -> Product3/1
  Sum2/1 -> Product1/2
  Constant3/1 -> Product1/3
  POT^3/1 -> lower limit 50/1
  Sum3/1 -> P40^3/1
  "upper limit 8  "/1 -> Sum3/1
  Constant7/1 -> Product4/1
  Sum4/1 -> Product4/2
  Product6/1 -> Sum4/2
  Constant8/1 -> Product6/1
  Manual Switch1/1 -> Product6/2
  Manual Switch2/1 -> Product7/1, Product6/3
  Sum6/1 -> Product6/4
  Integrator QO1/1 -> Sum4/1, Product2/2
  lower limit 50/1 -> Product1/1
  Sum1/1 -> Integrator QO2/1
  Integrator QO2/1 -> Product3/2
  Z2/1 -> Integrator QO2/2
  Z1/1 -> Integrator QO1/2
  Product4/1 -> Integrator QO1/1
  Product7/1 -> Sum6/2
  Product22/1 -> " VAS"/1
  Constant23/1 -> Product22/2
  Sum14/1 -> Product22/1
  Constant19/1 -> Sum15/2
  lower limit 0.2/1 -> Sum14/1
  Sum15/1 -> lower limit 0.2/1
  Sum13/1 -> Product19/1, Product17/1, Switch1/1, Product21/1, Switch1/2
  Constant25/1 -> Sum13/2
  Constant24/1 -> " VAS"/2
  " VAS"/1 -> Sum14/2, Product18/1
  Manual Switch121/1 -> Manual Switch61/2, Display2/1  "ARM"
  Product17/1 -> Sum16/1
  Product19/1 -> Sum15/1
  Constant26/1 -> Product19/2
  Constant27/1 -> Sum16/2
  Sum16/1 -> lower limit 0.5/1
  lower limit 0.5/1 -> Sum17/1
  Sum17/1 -> Product20/1
  Constant28/1 -> Product20/2
  Product20/1 -> " VAS1"/1
  Constant29/1 -> " VAS1"/2
  " VAS1"/1 -> Sum17/2, Product18/2
  Constant30/1 -> Product17/2
  Product21/1 -> Switch1/3
  POK8/1 -> Product21/2
  Switch1/1 -> Product23/1
  Constant31/1 -> Product23/2
  Product23/1 -> Sum18/1
  Sum18/1 -> lower limit 0.3/1
  lower limit 0.3/1 -> Sum19/1
  Constant20/1 -> Sum18/2
  Sum19/1 -> Product24/1
  Constant21/1 -> Product24/2
  Product24/1 -> " VAS2"/1
  Constant22/1 -> " VAS2"/2
  " VAS2"/1 -> Sum19/2, Product18/3
  Product27/1 -> Integrator/1
  Sum20/1 -> Product27/2
  Manual Switch58/1 -> Sum20/3, Display9/1, Manual Switch70/2
  Product26/1 -> Sum20/2
  Product25/1 -> Sum20/1
  Constant33/1 -> Product25/2, Product26/1
  Constant32/1 -> Product25/1
  SRK/1 -> Product27/1
  Manual Switch10/1 -> Sum25/2, Product43/2
  Constant47/1 -> Sum29/2
  Sum29/1 -> Product28/1
  ARF/1 -> Product28/2
  Product28/1 -> Sum21/1
  Constant35/1 -> Sum21/2
  Sum21/1 -> Product37/1
  Manual Switch13/1 -> Product38/2, Product37/2  "VIM"
  Constant40/1 -> Product37/4
  Product37/1 -> Product39/1, Sum24/1  "AAR"
  Constant41/1 -> Product38/1
  Sum24/1 -> " lower limit 0"/1  "RR"
  Manual Switch74/1 -> Display12/1  "RFN"
  Product39/1 -> Sum25/1
  Sum25/1 -> Sum26/2  "GLP"
  Manual Switch11/1 -> Sum26/3  "PPC"
  Constant42/1 -> Sum26/1
  Sum26/1 -> Product40/1  "PFL"
  Constant43/1 -> Product40/2
  Product40/1 -> Manual Switch25/2, Display72/1, Product41/1, Product42/2  "GFN"
  Constant44/1 -> Product42/1
  Constant45/1 -> Sum27/1
  Product42/1 -> Sum27/2
  GF4/1 -> Product44/1
  Sum27/1 -> Product44/2
  Sum28/1 -> upper limit 15.0 lower limit 0.4/1
  Product41/1 -> Product30/2, Sum30/1  "GFR"
  Constant36/1 -> Product30/1
  Sum31/1 -> Sum30/2  "TRR"
  Sum30/1 -> lower limit 0.0003/1  "VUD"
  Constant37/1 -> Product31/1
  Manual Switch76/1 -> Product31/2, Manual Switch78/2, Display10/1  "VUD"
  Constant38/1 -> Product32/1
  Constant39/1 -> Product33/2
  Product30/1 -> Sum31/1
  Sum22/1 -> Sum31/2  "TRR1"
  Product33/1 -> Sum22/2  "TRRMAX"
  Product32/1 -> Product34/1
  Manual Switch16/1 -> Product34/2, Display67/1  "AHM"
  Manual Switch17/1 -> Product34/3, Product36/1, Display66/1  "AM"
  Product34/1 -> Sum22/1  "NOREABS"
  CNX/1 -> Product35/2
  Manual Switch14/1 -> Product35/1
  Product31/1 -> Product36/2
  Manual Switch91/1 -> Display13/1, Manual Switch32/1  "NOD"
  CNY/1 -> Sum23/1
  Product35/1 -> Sum23/2
  Product38/1 -> Sum24/2  "EVR"
  Sum23/1 -> Product36/3
  Manual Switch59/1 -> Display11/1, Manual Switch67/2  "RBF"
  " lower limit 0.35"/1 -> Sum29/1
  Sum33/1 -> Product46/1
  Manual Switch92/1 -> Manual Switch33/1, Display20/1  "STH"
  "Z10 "/1 -> Sum33/2
  Product47/1 -> Sum32/1
  Constant48/1 -> Product47/2
  Constant49/1 -> Sum32/2
  Sum32/1 -> Product45/2
  Product45/1 -> lower limit 0/1
  lower limit 0/1 -> Display21/1, Manual Switch86/1
  "Z11 "/1 -> Product46/2
  Constant54/1 -> Sum38/2
  Constant52/1 -> Product51/1
  Product49/1 -> Math Function/1
  Integrator2/1 -> Product49/1, Sum34/2
  Constant55/1 -> Product49/2
  Constant56/1 -> Product50/1
  Sum35/1 -> lower limit 3/1
  lower limit 3/1 -> Product50/2
  Product52/1 -> Sum35/1
  CNR/1 -> Sum36/2
  Sum36/1 -> Product52/2  "CNB"
  Manual Switch20/1 -> Sum36/1
  Manual Switch19/1 -> Product53/1
  Constant59/1 -> Product53/2
  Product53/1 -> Sum37/2
  Sum37/1 -> Product48/1, Sum35/2
  Product48/1 -> Integrator1/1
  Integrator1/1 -> Sum37/1
  Constant60/1 -> Product48/2
  Constant61/1 -> Sum39/2
  Sum39/1 -> lower_limit_0/1
  lower_limit_0/1 -> Sum35/3
  Manual Switch94/1 -> Manual Switch16/2, Manual Switch22/2, Display22/1
  Product50/1 -> Sum34/1
  Constant58/1 -> Product52/1
  lower limit 0.95/1 -> Product77/1, Sum133/2, Display76/1, Sum134/1, Product55/1  "ANU"
  RAR/1 -> Product77/4  "RAR"
  Manual Switch64/1 -> lower limit 0.95/1
  Constant73/1 -> " VAS3"/2
  " VAS3"/1 -> Sum40/2, Sum62/1  "VAS"
  Constant80/1 -> Sum40/1
  Sum40/1 -> Product76/2  "VAE"
  Constant81/1 -> Product76/1  "CA"
  Manual Switch135/1 -> Sum51/1, Display60/1, Product66/2, Manual Switch10/2, Display63/1, Manual Switch27/2, Display69/1, Manual Switch40/1, Manual Switch55/1, Product57/1  "PA"
  Constant62/1 -> Product66/1
  Product66/1 -> Product77/6, Product55/6  "PAM"
  RAM/1 -> Product55/4
  Sum51/1 -> Product78/2, Product80/2  "PGS"
  Product77/1 -> Sum56/1
  Sum56/1 -> Product78/1  "RSN"
  Product55/1 -> Product80/1  "RSM"
  Manual Switch133/1 -> Display52/1, Sum57/3, Manual Switch2/2, Display61/1, Manual Switch80/1  "BFN"
  Manual Switch134/1 -> Manual Switch6/2, Sum57/2, Display53/1  "BFM"
  Product81/1 -> Sum56/2
  Sum57/1 -> Sum60/1, Sum61/2  "QAO"
  Manual Switch130/1 -> Product81/2, Display54/1, Manual Switch79/2
  CN2/1 -> Product63/2
  Sum58/1 -> Product63/1
  Constant68/1 -> Sum58/2
  Product65/1 -> Sum58/1
  CN7/1 -> Product65/2
  Constant69/1 -> Sum59/1
  Manual Switch68/1 -> Sum59/2
  Constant67/1 -> Product67/1
  " VVS"/1 -> Sum43/3, Sum62/6  "VVS"
  Manual Switch131/1 -> Sum44/2, Display8/1, Manual Switch9/1
  Sum44/1 -> lower limit 0.0001/1  "VV8"
  lower limit 0.0001/1 -> Product56/1
  CV/1 -> Product56/2
  Manual Switch129/1 -> Sum51/2, Sum48/2, Product68/1, Display55/1, Manual Switch81/2  "PVS"
  Product64/1 -> Sum60/3, Sum49/2  "QVO"
  Sum60/1 -> " VVS"/1  "DVS"
  Sum61/1 -> " VAS3"/1
  Manual Switch136/1 -> Manual Switch54/1, Sum61/1, Product60/1, Sum41/2, Display57/1  "QLO"
  LVM = f(PA2)/1(LVM) -> Product79/2
  QLN = f(PLA)/1(QLN) -> Product59/2, Product79/3  "QLN"
  Manual Switch72/1 -> Product61/6, Product79/5
  Manual Switch73/1 -> Product79/6
  Product57/1 -> LVM = f(PA2)/1(PA2)
  Constant82/1 -> " VLA"/2
  Sum41/1 -> " VLA"/1  "DLA"
  " VLA"/1 -> Sum42/2, Sum62/2  "VLA"
  Constant83/1 -> Sum42/1
  Sum42/1 -> Product58/2  "VLE"
  Constant63/1 -> Product58/1
  Manual Switch137/1 -> Sum54/2, Sum53/1, QLN = f(PLA)/1(PLA), Display58/1, Manual Switch48/2  "PLA"
  Manual Switch75/1 -> Sum62/5  "VB"
  Product60/1 -> Product59/1
  QRF/1 -> Product60/2, Sum45/1
  "1 "/1 -> Sum45/2
  RVM = f(PP2)/1(RVM) -> Product61/1  "RVM"
  Sum45/1 -> Product61/3
  Product61/1 -> Sum46/2
  Product59/1 -> Sum46/1
  QRN = f(PRA)/1(QRN) -> Product62/2  "QRN"
  Sum46/1 -> Product62/1
  Product62/1 -> Sum47/2, Sum49/1
  Constant79/1 -> Product68/2
  Product68/1 -> Product64/1  "RVG"
  Sum48/1 -> Product64/2
  Constant85/1 -> " VRA"/2
  Sum49/1 -> " VRA"/1  "DRA"
  " VRA"/1 -> Sum52/1, Sum62/4  "VRA"
  Constant64/1 -> Sum52/2
  Sum52/1 -> Product69/2
  Constant65/1 -> Product69/1
  Manual Switch132/1 -> lower limit = 0/1, Display56/1, Manual Switch19/2, Manual Switch53/1, QRN = f(PRA)/1(PRA)  "PRA"
  lower limit = 0/1 -> Sum48/1  "PR1"
  Constant66/1 -> " VPA"/2
  Sum47/1 -> " VPA"/1
  Product70/1 -> RVM = f(PP2)/1(PP2)  "PP2"
  " VPA"/1 -> Sum50/1, Sum62/3  "VPA"
  Constant71/1 -> Sum50/2
  Sum50/1 -> Product71/1
  Constant72/1 -> Product71/2
  Manual Switch138/1 -> Product70/2, Product74/2, Display59/1, Manual Switch47/1, Manual Switch41/1, Sum53/2
  Sum53/1 -> Product72/2  "PGL"
  Product72/1 -> Sum41/1, Sum47/1  "QPO"
  Constant74/1 -> Sum54/1
  Constant76/1 -> Product73/1
  Sum54/1 -> Product73/2
  Constant75/1 -> Product73/3
  Constant77/1 -> Product74/1
  Product73/1 -> Sum55/1
  Sum55/1 -> Product72/1
  Product75/1 -> Sum55/2  "RPA"
  Constant78/1 -> Product75/1
  Math Function1/1 -> Product75/2  "CPA"
  Product74/1 -> "lower limit 0 "/1
  "lower limit 0 "/1 -> Math Function1/1
  Sum62/1 -> Sum60/2
  Constant70/1 -> " VVS"/2
  Manual Switch79/1 -> Product84/1
  Constant92/1 -> Product84/2
  Manual Switch80/1 -> Product84/3
  Product84/1 -> Sum64/2
  Manual Switch81/1 -> Sum64/1
  Manual Switch125/1 -> Sum63/3, Manual Switch68/1, Display30/1, PC^3/1
  Manual Switch123/1 -> Sum63/4, Display35/1, Manual Switch49/1, Manual Switch11/2, Display64/1
  Constant86/1 -> Product83/2
  Manual Switch128/1 -> Sum67/1, Display34/1, Manual Switch50/1, Sum69/2, Product83/1  "CPP"
  Manual Switch126/1 -> Manual Switch75/1, Manual Switch46/1
  Manual Switch84/1 -> Sum63/1
  Manual Switch83/1 -> Sum63/2
  Manual Switch82/1 -> Sum65/1
  Sum63/1 -> Product85/2
  CFC/1 -> Product85/1
  Z6/1 -> "KE "/2
  Sum66/1 -> "KE "/1
  Manual Switch85/1 -> Sum66/4
  Manual Switch86/1 -> Sum66/1  "TVD"
  Manual Switch87/1 -> Sum66/5
  Manual Switch122/1 -> Product89/2, Sum65/2, Display32/1, Manual Switch35/2
  PC^3/1 -> Product86/1
  CPK/1 -> Product86/2
  Sum67/1 -> Product87/1
  Manual Switch89/1 -> Sum67/2
  KE 1/1 -> Product89/1  "PRP"
  Z5/1 -> KE 1/2
  Sum68/1 -> KE 1/1
  DP0/1 -> Sum68/3
  Constant90/1 -> Sum69/1
  Sum69/1 -> Product88/1
  LPK/1 -> Product88/2
  Manual Switch88/1 -> Sum68/1
  Manual Switch90/1 -> Sum68/4
  Product86/1 -> Product87/2
  Manual Switch127/1 -> Sum68/5, Manual Switch39/2, Display33/1
  Product88/1 -> Sum68/2  "DLP"
  Manual Switch124/1 -> Sum66/2, Manual Switch37/2, Display36/1  "VTC"
  Manual Switch24/1 -> Sum70/1, Product166/2
  Constant93/1 -> Sum70/2
  Sum71/1 -> Product93/1
  Constant95/1 -> Product93/2  "ANT"
  Product93/1 -> Integrator3/1
  Integrator3/1 -> Sum71/1, Product92/2  "ANC"
  Product92/1 -> Math Function2/1
  Constant96/1 -> Product92/1
  Math Function2/1 -> Product94/2
  Constant97/1 -> Product94/1
  Product94/1 -> Sum72/1
  Constant98/1 -> Sum72/2
  Sum72/1 -> lower limit 0.7/1
  Manual Switch95/1 -> Manual Switch64/1, Manual Switch26/2, Display23/1  "ANM"
  Xo2/1 -> Integrator3/2
  Constant101/1 -> Product104/1
  Manual Switch104/1 -> Manual Switch90/1, Display38/1, Sum81/2
  Sum81/1 -> KE 3/1
  IFP0/1 -> KE 3/2
  KE 3/1 -> Product106/1  "IFP"
  Manual Switch105/1 -> Product104/2, Product96/2, Display40/1, Manual Switch89/2, Sum77/1
  Sum77/1 -> Product101/2
  Product101/1 -> Product102/2
  Constant99/1 -> Product102/1
  Product102/1 -> Sum81/3, KE 2/1
  KE 2/1 -> Product103/2
  Product105/1 -> lower limit =  0/1
  Sum73/1 -> Product105/1
  Constant103/1 -> Product105/2
  Constant102/1 -> Sum73/3
  Manual Switch103/1 -> Manual Switch87/1, Display37/1, Sum79/2
  Manual Switch37/1 -> Sum79/1
  Manual Switch106/1 -> Display39/1, Manual Switch84/1, Sum80/2
  Manual Switch39/1 -> Sum81/1
  PTS = f(VIF)/1(AMP) -> Sum74/2, Sum76/1
  Manual Switch102/1 -> Sum74/1, Sum80/3, Sum73/1, Manual Switch83/1, Display42/1
  Manual Switch101/1 -> Sum78/1, Manual Switch36/2, PTT = (VTS/12)^2/1, Display41/1  "VTS"
  PTT = (VTS/12)^2/1 -> Sum76/2, Sum73/2
  Sum78/1 -> PTS = f(VIF)/1(VIF), Product106/2  "VIF"
  KE 5/1 -> Sum78/2, Product97/1, Product101/1, Product103/1  "VG"
  Z10/1 -> KE 5/2
  Product107/1 -> KE 5/1  "VGD"
  Constant104/1 -> Product107/1
  Sum82/1 -> Sum80/1
  Product108/1 -> Sum82/1
  Constant105/1 -> Product108/1
  Constant106/1 -> Product97/2
  Product97/1 -> Product108/2, CHY^2/1, Product98/1
  Constant107/1 -> Product98/2
  Product98/1 -> Sum83/1
  Constant108/1 -> Sum83/2
  Sum83/1 -> Sum74/3
  Sum74/1 -> Sum80/4
  Product99/1 -> Sum82/2
  Sum75/1 -> Product99/1, Sum77/2
  Constant109/1 -> Product99/2
  Product103/1 -> Sum75/2, Product100/2
  Product100/1 -> Sum75/1
  Constant100/1 -> Product100/3
  CHY^2/1 -> Product100/1
  Manual Switch38/1 -> Sum79/3
  Sum79/1 -> KE 4/1
  Z9/1 -> KE 4/2
  Z7/1 -> KE 2/2
  Sum80/1 -> Product107/2
  Manual Switch28/1 -> Product112/2
  Constant115/1 -> Product112/1
  Manual Switch29/1 -> Product112/3
  Constant110/1 -> Sum84/2
  Product112/1 -> Sum84/1
  Sum84/1 -> lower limit 6/1
  lower limit 6/1 -> Product110/3
  Manual Switch26/1 -> Product110/1
  Product110/1 -> Sum85/1
  Sum85/1 -> Product109/2
  Constant111/1 -> Product109/1
  KE 6/1 -> Product111/2, Sum85/2
  Constant112/1 -> Product111/1
  Product111/1 -> Math Function3/1
  Math Function3/1 -> Product113/2
  Constant113/1 -> Product113/1
  Product113/1 -> Sum86/2
  Constant114/1 -> Sum86/1
  Manual Switch97/1 -> Manual Switch17/2, Manual Switch30/2, Display25/1
  Manual Switch27/1 -> AMP = f(PA)/1(PA)
  AMP = f(PA)/1(AMP) -> Product110/2
  Product109/1 -> KE 6/1
  Z11/1 -> KE 6/2
  Manual Switch36/1 -> Sum87/3  "VTS"
  Manual Switch35/1 -> Sum87/2  "VP"
  Manual Switch34/1 -> Sum87/1
  Sum87/1 -> Product114/2, Product120/2, Sum88/2  "VEC"
  Sum88/1 -> Display29/1  "VTW"
  Manual Switch33/1 -> Product119/1  "STH2NID"
  Manual Switch142/1 -> Product119/2  "NID"
  Product119/1 -> Sum89/2  "NID2"
  Sum89/1 -> Integrator QO6/1  "NED"
  Integrator QO6/1 -> Product114/1  "NAE"
  Sum90/1 -> Product116/1
  Product117/1 -> Sum90/1
  Constant117/1 -> Product117/2
  Product118/1 -> Sum90/2
  Constant118/1 -> Product118/1
  Manual Switch99/1 -> Product118/3, Product122/1, Display27/1, Manual Switch28/2, Display71/1, Product117/1
  Constant119/1 -> Sum91/2
  Product116/1 -> Sum91/3
  Manual Switch30/1 -> Product118/2
  Product121/1 -> Integrator QO5/1, Sum91/1
  Sum92/1 -> Product121/1
  Constant120/1 -> Product121/2
  Sum93/1 -> Sum92/2
  Product122/1 -> Sum93/2
  Constant121/1 -> Product122/2
  Integrator QO5/1 -> Sum92/1, Product123/1
  Product123/1 -> Sum94/1
  Sum94/1 -> Product115/1
  Constant122/1 -> Product115/2
  Z14/1 -> Integrator QO7/2
  Manual Switch98/1 -> Display26/1, Manual Switch38/2
  Integrator QO7/1 -> Sum88/1, Product123/2
  Manual Switch100/1 -> Display28/1, Sum94/2, Manual Switch24/2, Manual Switch20/2, Manual Switch29/2, Display70/1  "CNA"
  Constant123/1 -> Sum93/1
  Z13/1 -> Integrator QO6/2
  Z15/1 -> KE 7/2
  KE 7/1 -> Product120/1
  Sum91/1 -> KE 7/1
  Z12/1 -> Integrator QO5/2
  Manual Switch40/1 -> Product128/2
  Constant124/1 -> Product128/3
  Product128/1 -> PA4^0.625/1
  PA4^0.625/1 -> Sum97/1
  Sum97/1 -> Product124/1
  Constant125/1 -> Product124/2
  Product124/1 -> KE 8/1
  Z18/1 -> KE 8/2
  Manual Switch109/1 -> Sum97/2, Display44/1, Manual Switch73/2
  Manual Switch41/1 -> Product125/2
  Constant126/1 -> Product125/3
  Product125/1 -> PP3^0.1/1
  PP3^0.1/1 -> Sum95/1
  Sum95/1 -> Product126/1
  Z16/1 -> KE 9/2
  Product126/1 -> KE 9/1
  Constant127/1 -> Product126/2
  Manual Switch108/1 -> Sum95/2, Display43/1, Manual Switch77/2
  Constant128/1 -> Sum96/2
  Sum96/1 -> Product127/1
  Constant129/1 -> Product127/2
  Product127/1 -> KE 10/1
  Z17/1 -> KE 10/2
  KE 10/1 -> upper limit 1/1
  Manual Switch107/1 -> Display45/1, Manual Switch72/2, Manual Switch52/1
  PO1/1 -> Sum100/1
  Sum100/1 -> lower limit 0.2375/1
  lower limit 0.2375/1 -> Product133/1
  POY/1 -> Product133/2
  Product133/1 -> Sum98/2
  Sum98/1 -> KE 11/1
  Z20/1 -> KE 11/2
  Manual Switch110/1 -> Product129/1, Display48/1, Manual Switch82/1, Product134/1
  Constant131/1 -> Product129/2
  Product129/1 -> Sum98/1
  Manual Switch46/1 -> Product134/2  "VB"
  Product134/1 -> Product130/2
  Constant132/1 -> Product130/1
  Manual Switch111/1 -> Display47/1, Manual Switch5/2, Manual Switch1/2, Sum101/2, Product131/1  "HM"
  Constant134/1 -> Product135/1
  Product135/1 -> Sum99/2
  Constant135/1 -> Sum99/1
  Sum99/1 -> Product132/2
  Constant136/1 -> Product132/1
  Manual Switch112/1 -> Display46/1, Manual Switch62/2, Manual Switch13/2, Display73/1
  Manual Switch47/1 -> Product136/1
  Constant140/1 -> Product136/2
  Product136/1 -> Sum103/1
  Product137/1 -> Sum103/2
  Constant138/1 -> Product137/1
  Manual Switch48/1 -> Product137/2
  Sum103/1 -> Sum102/1
  Manual Switch49/1 -> Sum102/2
  CPF/1 -> Product138/2
  Product138/1 -> Sum104/1
  Constant139/1 -> " VAS5"/2
  Manual Switch115/1 -> Display49/1, Manual Switch85/1, " VAS5"/1
  Manual Switch114/1 -> PPI = 2 - (0.15/VPF)/1, Product142/2, Display50/1, Manual Switch4/2, Manual Switch34/2
  PPI = 2 - (0.15/VPF)/1 -> Sum102/4, Sum105/2
  Constant142/1 -> Sum105/1
  Sum105/1 -> Product139/2
  Constant143/1 -> Product139/1
  Product139/1 -> Product143/1, Sum104/2
  Sum107/1 -> Product140/2
  Constant144/1 -> Product140/1
  Manual Switch50/1 -> Sum107/1
  Product140/1 -> Sum106/1
  Manual Switch113/1 -> " VAS4"/1, Display51/1, Manual Switch88/1
  Constant145/1 -> " VAS4"/2
  " VAS4"/1 -> Product142/1
  Product142/1 -> Product141/2, Sum107/2, Product143/2
  Constant146/1 -> Product141/1
  Product141/1 -> Sum102/3
  Product143/1 -> Sum106/2
  Sum102/1 -> Product138/1
  Product151/1 -> Sum113/1
  Constant147/1 -> Product151/2
  Product147/1 -> Product151/1
  upper limit 8 lower limit 4/1 -> Product147/1
  Manual Switch55/1 -> Product147/2
  Sum108/1 -> Sum113/2
  Product144/1 -> Sum108/1
  Constant156/1 -> Product144/1
  Sum114/1 -> Product144/2
  Constant157/1 -> Sum114/1
  Product146/1 -> Sum108/2
  Sum115/1 -> Product146/1
  Constant158/1 -> Sum115/2
  Constant159/1 -> Product146/2
  Sum113/1 -> AUC calculation/1(PA1), AUN calculation/1(PA1), AUB calculation/1(PA1)
  AUC calculation/1(AUC) -> Sum116/3
  AUB calculation/1(AUB) -> AUB^3/1
  AUB^3/1 -> Sum117/1
  Sum117/1 -> Sum118/1, Sum116/2
  Constant160/1 -> Sum118/2
  Sum118/1 -> Product148/2
  Constant161/1 -> Product148/1
  KE 13/1 -> Sum117/2
  Z21/1 -> KE 13/2
  Product148/1 -> KE 13/1
  AUN calculation/1(AUN) -> Sum116/1
  Sum116/1 -> Sum119/2
  Sum119/1 -> Product149/1
  Z8/1 -> Product149/2
  Product149/1 -> KE 14/1
  Z22/1 -> KE 14/2
  KE 14/1 -> Sum119/1, AUJ^AUZ/1
  Product150/1 -> Sum120/2
  VV9/1 -> Sum120/1
  Manual Switch119/1 -> Manual Switch69/1, Display15/1
  AUV/1 -> Product152/2
  Product152/1 -> Sum109/2
  Manual Switch71/1 -> Product57/2, Product79/4, Product61/2, Product70/1
  Product153/1 -> Sum110/1
  Constant151/1 -> Sum110/2
  Constant152/1 -> Product153/2
  Manual Switch117/1 -> Sum111/2, Manual Switch63/1, Manual Switch15/1, Display65/1, Display17/1
  Constant153/1 -> Sum111/1
  Sum111/1 -> Product145/2
  AUY/1 -> Product145/1
  Product145/1 -> Sum112/2
  Manual Switch116/1 -> Display18/1, Manual Switch66/2
  Constant155/1 -> Sum112/1
  Manual Switch54/1 -> Product158/1
  Product154/1 -> Product158/2, Display62/1  "HR"
  Sum122/1 -> Product154/1
  Constant168/1 -> Sum122/1
  Product157/1 -> Sum122/2
  Constant164/1 -> Product157/1
  Manual Switch53/1 -> Product157/2
  Constant165/1 -> Product155/1
  Product155/1 -> Sum122/3
  Manual Switch52/1 -> Sum123/1
  Constant166/1 -> Sum123/2
  Sum123/1 -> Product156/1
  Constant167/1 -> Product156/2
  Product156/1 -> Sum121/2
  Sum121/1 -> Product154/2
  Constant169/1 -> Sum121/1
  Product15/1 -> Sum124/1
  Sum124/1 -> Product162/1
  Constant10/1 -> Product162/4
  Manual Switch23/1 -> Product15/1, Display3/1, Manual Switch3/1
  Manual Switch5/1 -> Product162/3, Product9/2
  Constant172/1 -> Product9/3
  Sum7/1 -> Product9/1
  Constant176/1 -> Sum7/2
  Product14/1 -> Sum7/1
  Constant177/1 -> Product14/2
  Manual Switch6/1 -> Product15/2, Product162/2
  Manual Switch4/1 -> Product14/1
  Product162/1 -> Sum125/2
  Sum125/1 -> Product16/1
  Constant178/1 -> Product16/2
  Product16/1 -> Integrator4/1
  Integrator4/1 -> Sum125/1, Product159/1  "OVS"
  Constant179/1 -> Product159/2
  Product159/1 -> Sum126/1, Sum9/2
  Sum126/1 -> Product160/1
  Constant180/1 -> Product160/2
  Product160/1 -> Sum124/2, Sum127/1
  Integrator7/1 -> Sum128/2
  Constant181/1 -> Sum128/1
  Sum128/1 -> Product161/2
  Constant182/1 -> Product161/1
  lower limit .001/1 -> PM1^2/1
  Constant11/1 -> Sum129/2
  PM1^2/1 -> Sum129/1
  Manual Switch31/1 -> Sum130/1, Manual Switch57/1, Display4/1
  Sum130/1 -> P3O^3/1
  Constant12/1 -> Sum130/2
  P3O^3/1 -> Product163/1
  Constant13/1 -> Product163/2
  Product163/1 -> Sum131/2
  Constant14/1 -> Sum131/1
  Sum131/1 -> Product10/2  "PDOM"
  Constant15/1 -> Product10/1
  Constant190/1 -> Product10/3, Sum115/1
  Product10/1 -> Sum127/2  "MMO"
  Constant16/1 -> Sum10/2
  Product11/1 -> Sum10/1
  Constant17/1 -> Product11/1
  Sum11/1 -> Product11/2
  Constant18/1 -> Sum11/1
  Product12/1 -> Integrator5/1
  Constant170/1 -> Product12/1
  Sum12/1 -> Product12/2
  Sum8/1 -> lower limit .005/1
  Constant171/1 -> Sum8/1
  Product13/1 -> Sum8/2
  Sum9/1 -> Product13/2
  Constant173/1 -> Product13/1
  Constant174/1 -> Sum9/1
  Manual Switch43/1 -> Product10/4, Display6/1, Manual Switch/1
  lower limit .005/1 -> Sum12/1
  Product161/1 -> lower limit .001/1, Sum126/2, upper limit 8/1
  Sum127/1 -> Integrator7/1
  Xo/1 -> Integrator7/2
  Sum129/1 -> Product160/3
  Xo1/1 -> Integrator5/2
  Manual Switch42/1 -> Sum12/2, Display7/1, Manual Switch65/2
  Xo3/1 -> Integrator4/2
  Product158/1 -> Display19/1  "SVO"
  Manual Switch/1 -> Product5/1
  Constant183/1 -> Manual Switch/2
  Constant184/1 -> Manual Switch1/1
  Constant185/1 -> Manual Switch2/1
  Manual Switch3/1 -> Product7/2
  Constant186/1 -> Manual Switch3/2
  Constant187/1 -> Manual Switch4/1
  Constant188/1 -> Manual Switch5/1
  Constant189/1 -> Manual Switch6/1
  Manual Switch8/1 -> Sum11/2
  Constant191/1 -> Manual Switch8/2
  Manual Switch9/1 -> Product26/2
  Constant192/1 -> Manual Switch9/2
  Constant193/1 -> Manual Switch10/1
  Constant194/1 -> Manual Switch11/1
  Manual Switch143/1 -> Product116/2, Product95/1, Product41/2, Product29/2, Product32/2, Product33/1  "REK"
  Constant196/1 -> Manual Switch13/1
  Constant197/1 -> Manual Switch14/1
  Manual Switch15/1 -> " lower limit 0.35"/1
  Constant198/1 -> Manual Switch15/2
  Constant199/1 -> Manual Switch16/1
  Constant200/1 -> Manual Switch17/1
  Manual Switch18/1 -> Sum39/1  "AU"
  Constant201/1 -> Manual Switch18/2
  Constant202/1 -> Manual Switch19/1
  Constant203/1 -> Manual Switch20/1
  Constant204/1 -> Manual Switch21/1
  Manual Switch21/1 -> Sum33/1
  Constant205/1 -> Manual Switch22/1
  Manual Switch22/1 -> Product47/1
  Constant207/1 -> Manual Switch24/1
  Constant208/1 -> Manual Switch25/1
  Constant209/1 -> Manual Switch26/1
  Constant210/1 -> Manual Switch27/1
  Constant211/1 -> Manual Switch28/1
  Constant212/1 -> Manual Switch29/1
  Constant213/1 -> Manual Switch30/1
  Manual Switch32/1 -> Sum89/1
  Constant215/1 -> Manual Switch32/2
  Constant217/1 -> Manual Switch34/1
  Constant218/1 -> Manual Switch35/1
  Constant219/1 -> Manual Switch36/1
  Constant220/1 -> Manual Switch37/1
  Constant221/1 -> Manual Switch38/1
  Constant222/1 -> Manual Switch39/1
  Constant223/1 -> Manual Switch40/2
  Constant224/1 -> Manual Switch41/2
  Manual Switch44/1 -> Sum96/1
  Constant227/1 -> Manual Switch44/1
  Manual Switch45/1 -> Sum100/2
  Constant228/1 -> Manual Switch45/1
  Constant229/1 -> Manual Switch46/2
  Constant230/1 -> Manual Switch47/2
  Constant231/1 -> Manual Switch48/1
  Constant232/1 -> Manual Switch49/2
  Constant233/1 -> Manual Switch50/2
  Constant234/1 -> Manual Switch51/2
  Manual Switch51/1 -> Product155/2
  Constant235/1 -> Manual Switch52/2
  Constant236/1 -> Manual Switch53/2
  Constant237/1 -> Manual Switch54/2
  Constant238/1 -> Manual Switch55/2
  Constant239/1 -> Manual Switch56/2
  Manual Switch56/1 -> upper limit 8 lower limit 4/1
  Constant240/1 -> Manual Switch57/2
  Manual Switch57/1 -> Sum114/2
  AUZ/1 -> AUJ^AUZ/2
  Manual Switch60/1 -> Sum13/1
  Constant243/1 -> Manual Switch60/1
  Constant244/1 -> Manual Switch61/1
  Manual Switch61/1 -> Product77/2
  Constant245/1 -> Manual Switch62/1
  Constant246/1 -> Manual Switch63/2
  Manual Switch63/1 -> Product77/5, Product55/5
  Constant247/1 -> Manual Switch64/2
  Constant248/1 -> Manual Switch65/1
  Manual Switch65/1 -> Product55/2
  Constant249/1 -> Manual Switch66/1
  Constant250/1 -> Manual Switch67/1
  Manual Switch67/1 -> Sum57/1  "RBF"
  Constant251/1 -> Manual Switch68/2
  Constant252/1 -> Manual Switch69/2
  Constant253/1 -> Manual Switch70/1
  Manual Switch70/1 -> Sum44/1
  Constant254/1 -> Manual Switch71/1
  Manual Switch118/1 -> Display16/1, Manual Switch71/2  "AUH"
  Constant255/1 -> Manual Switch72/1
  Constant256/1 -> Manual Switch73/1
  Constant257/1 -> Product79/1, Manual Switch139/1
  Constant258/1 -> Manual Switch75/2
  Constant260/1 -> Manual Switch77/1
  Manual Switch77/1 -> Product61/5
  Constant216/1 -> Manual Switch33/2
  Constant261/1 -> Manual Switch78/1
  Manual Switch78/1 -> Sum66/3  "VUD"
  Constant262/1 -> Manual Switch79/1
  Constant263/1 -> Manual Switch80/2
  Constant264/1 -> Manual Switch81/1
  Constant265/1 -> Manual Switch82/2
  Constant266/1 -> Manual Switch83/2
  Constant267/1 -> Manual Switch84/2
  Constant268/1 -> Manual Switch85/2
  Constant269/1 -> Manual Switch86/2
  Constant270/1 -> Manual Switch87/2
  Constant271/1 -> Manual Switch88/2
  Constant272/1 -> Manual Switch89/1
  Constant273/1 -> Manual Switch90/2
  " lower limit 0"/1 -> Product43/1
  Product164/1 -> Integrator2/1
  Constant53/1 -> Product164/2
  HSR/1 -> Product61/4, Manual Switch140/1
  Manual Switch7/1 -> Display5/1, Manual Switch60/2
  Product2/1 -> Sum2/2, Manual Switch7/1
  Constant206/1 -> Manual Switch7/2
  Manual Switch12/1 -> POT^3/1, Sum2/1, "upper limit 8  "/1, Manual Switch44/2, Manual Switch45/2, Manual Switch56/1, Manual Switch21/2, Display1/1  "POT"
  Product3/1 -> Manual Switch12/1
  Constant214/1 -> Manual Switch12/2
  Product9/1 -> Manual Switch23/1
  Constant225/1 -> Manual Switch23/2
  upper limit 8/1 -> Manual Switch31/1
  Constant226/1 -> Manual Switch31/2
  Integrator5/1 -> Manual Switch42/1
  Constant241/1 -> Manual Switch42/2
  Sum10/1 -> Manual Switch43/2
  Constant274/1 -> Manual Switch43/1
  Integrator/1 -> Manual Switch58/1
  Constant275/1 -> Manual Switch58/2
  lower limit 0.0003/1 -> Manual Switch76/1
  Constant276/1 -> Manual Switch76/2
  Product36/1 -> Manual Switch91/1
  Constant277/1 -> Manual Switch91/2
  Product29/1 -> Manual Switch59/1
  Constant278/1 -> Manual Switch59/2
  Product43/1 -> Product39/2, Manual Switch74/1, Product29/1  "RFN"
  Constant279/1 -> Manual Switch74/2
  Product46/1 -> Manual Switch92/1, Product45/1
  Constant280/1 -> Manual Switch92/2
  Constant282/1 -> Manual Switch94/1
  lower limit 0.7/1 -> Manual Switch95/2
  Constant283/1 -> Manual Switch95/1
  Sum70/1 -> Manual Switch96/2
  Constant284/1 -> Manual Switch96/1
  Sum86/1 -> Manual Switch97/2
  Constant285/1 -> Manual Switch97/1
  Product114/1 -> Manual Switch100/1
  Constant288/1 -> Manual Switch100/2
  Product120/1 -> Manual Switch99/2
  Constant287/1 -> Manual Switch99/1
  Product115/1 -> Integrator QO7/1, Manual Switch98/2
  Constant286/1 -> Manual Switch98/1
  Constant289/1 -> Manual Switch101/1
  KE 4/1 -> Manual Switch101/2
  Product104/1 -> Manual Switch106/2
  Constant290/1 -> Manual Switch106/1
  Constant291/1 -> Manual Switch103/2
  Product106/1 -> Manual Switch105/1
  Constant294/1 -> Manual Switch105/2
  Product96/1 -> Manual Switch104/1
  Constant292/1 -> Manual Switch104/2
  Sum76/1 -> Manual Switch102/2
  Constant293/1 -> Manual Switch102/1
  upper limit 1/1 -> Manual Switch107/1
  Constant295/1 -> Manual Switch107/2
  KE 9/1 -> Manual Switch108/1
  Constant296/1 -> Manual Switch108/2
  KE 8/1 -> Manual Switch109/1
  Constant297/1 -> Manual Switch109/2
  KE 11/1 -> Manual Switch110/1
  Constant298/1 -> Manual Switch110/2
  Product132/1 -> Manual Switch112/2
  Constant299/1 -> Manual Switch112/1
  Product130/1 -> Manual Switch111/2
  Constant300/1 -> Manual Switch111/1
  Sum106/1 -> Manual Switch113/1
  Constant303/1 -> Manual Switch113/2
  " VAS5"/1 -> Manual Switch114/1
  Constant301/1 -> Manual Switch114/2
  Sum104/1 -> Manual Switch115/1
  Constant302/1 -> Manual Switch115/2
  Sum112/1 -> Manual Switch116/1
  Constant304/1 -> Manual Switch116/2
  Sum110/1 -> Manual Switch117/1  "AUM"
  Constant305/1 -> Manual Switch117/2
  Sum109/1 -> Manual Switch118/1
  Constant306/1 -> Manual Switch118/2
  Sum120/1 -> Manual Switch119/1
  Constant307/1 -> Manual Switch119/2
  Product18/1 -> Manual Switch121/2
  Constant309/1 -> Manual Switch121/1
  Product83/1 -> Manual Switch123/1
  Constant316/1 -> Manual Switch123/2
  "KE "/1 -> Manual Switch122/1
  Constant310/1 -> Manual Switch122/2
  Product89/1 -> Manual Switch128/2
  Constant311/1 -> Manual Switch128/1
  Product87/1 -> Manual Switch127/1
  Constant312/1 -> Manual Switch127/2
  Product85/1 -> Manual Switch124/2
  Constant313/1 -> Manual Switch124/1
  Sum64/1 -> Manual Switch125/1
  Constant314/1 -> Manual Switch125/2
  Sum65/1 -> Manual Switch126/2, Display31/1
  Constant315/1 -> Manual Switch126/1
  Product56/1 -> Manual Switch129/1
  Constant317/1 -> Manual Switch129/2
  Product82/1 -> Manual Switch130/1
  Constant318/1 -> Manual Switch130/2
  Sum43/1 -> Manual Switch131/1
  Constant319/1 -> Manual Switch131/2
  Product69/1 -> Manual Switch132/1
  Constant320/1 -> Manual Switch132/2
  Product78/1 -> Manual Switch133/1
  Constant321/1 -> Manual Switch133/2
  Product80/1 -> Manual Switch134/2
  Constant322/1 -> Manual Switch134/1
  Product76/1 -> Manual Switch135/1
  Constant323/1 -> Manual Switch135/2
  Product79/1 -> Manual Switch136/2
  Constant324/1 -> Manual Switch136/1
  Product58/1 -> Manual Switch137/2
  Constant325/1 -> Manual Switch137/1
  Product71/1 -> Manual Switch138/1
  Constant326/1 -> Manual Switch138/2
  upper limit 15.0 lower limit 0.4/1 -> Product37/3  "GF3"
  Product44/1 -> Sum28/1
  Constant46/1 -> Sum28/2
  Manual Switch139/1 -> Product128/1
  Constant327/1 -> Manual Switch139/2
  Constant328/1 -> Manual Switch140/2
  Manual Switch140/1 -> Product125/1
  Product131/1 -> Product135/2
  Z3/1 -> Sum101/1
  Sum101/1 -> Product131/2
  Sum34/1 -> Product164/1
  Xo6/1 -> Integrator1/2
  From Workspace/1 -> Manual Switch142/2
  Constant116/1 -> Manual Switch142/1
  Constant195/1 -> Manual Switch143/1
  From Workspace1/1 -> Manual Switch143/2
  lower limit =  0/1 -> Product96/1, Manual Switch103/1
  Constant84/1 -> Product81/1
  Sum134/1 -> Product54/1
  Manual Switch69/1 -> Sum43/2
  Product54/1 -> Sum43/1
  ANY/1 -> Product54/2
  Constant137/1 -> Sum134/2
  Sum59/1 -> Product65/1
  Product63/1 -> Display75/1, Product67/2  "CN3"
  Manual Switch66/1 -> Product82/3
  Product67/1 -> Product82/4  "RV1"
  Constant175/1 -> Sum133/1
  ANZ/1 -> Product165/1
  Sum133/1 -> Product165/2
  Manual Switch62/1 -> Product77/3, Product82/2, Product55/3
  Manual Switch96/1 -> Display24/1, Manual Switch14/2, Display68/1
  Manual Switch25/1 -> Product166/1
  Product166/1 -> Sum135/2
  Constant281/1 -> Sum135/1
  Sum135/1 -> Product167/2
  Product167/1 -> Sum136/2
  Constant329/1 -> Product167/1
  Constant330/1 -> Sum136/1
  Sum136/1 -> Product95/2
  Constant331/1 -> Sum137/2
  Sum137/1 -> Product168/2
  Constant332/1 -> Product168/1
  Product95/1 -> Sum139/1, Sum137/1  "ANP"
  Sum138/1 -> Product169/1
  Constant333/1 -> Product169/2
  Xo5/1 -> Integrator8/2
  Product169/1 -> Integrator8/1
  Product168/1 -> Sum138/2
  Integrator8/1 -> Sum139/2, Sum138/1
  Product165/1 -> Sum140/2
  Constant334/1 -> Sum140/1
  Sum140/1 -> Product82/1
  Sum139/1 -> lower limit = 0.01 upper limit =100/1
  lower limit = 0.01 upper limit =100/1 -> Sum71/2
  Manual Switch120/1 -> Display14/1, Manual Switch8/1, Manual Switch18/1
  Constant94/1 -> Sum141/1
  Sum141/1 -> Product152/1, Product91/1, Product90/1
  AUQ/1 -> Product90/2
  Product90/1 -> Sum142/2
  Constant335/1 -> Sum142/1
  Sum142/1 -> Product150/2, Product153/1
  Constant308/1 -> Manual Switch120/2
  AUJ^AUZ/1 -> Sum141/2, Manual Switch120/1
  AUL/1 -> Product150/1
  Constant149/1 -> Sum109/1
  AUS/1 -> Product91/2
  Constant150/1 -> Manual Switch93/2
  Manual Switch93/1 -> Manual Switch51/1, Display74/1
  Product91/1 -> Sum143/2
  Sum143/1 -> Manual Switch93/1
  Constant154/1 -> Sum143/1
  Product51/1 -> Manual Switch94/2
  Sum38/1 -> Product51/2
  Math Function/1 -> Sum38/1
